simulink model "SuspensionModel"  (R2023a)
settings: Solver=FixedStepAuto  StartTime=0.0  StopTime=30  FixedStep=1e-3  RelTol=1e-3
model workspace (MAT data in the model file):
  A = [0  1  0  -1; -444.444444444  -26.3931623932  0  26.3931623932; 0  0  0  1; 2418.60465116  143.627906977  -9302.3255814  -143.627906977]
  A_eso = [0  1  0; 0  0  1; 0  0  0]
  B = [0  0; 0  0.0042735042735; -1  0; 0  -0.0232558139535]
  B_eso_th = [0; 333.333333333; 0]
  B_eso_y = [0; 0.8; 0]
  C = [1  0  0  0; 0  1  0  0; 0  0  1  0; 0  0  0  1; -444.444444444  -26.3931623932  0  26.3931623932]
  C_eso = [1 0 0]
  D = [0  0; 0  0; 0  0; 0  0; 0  0.0042735042735]
  I = 0.003
  Ic_xnl = [0; 0; 0; 0; 0.349065850399; 0]
  Iyy = 2100
  K = [40277.510375 6943.43713521 -89611.1366666 302.327568335]
  Kd = 5239.23468894
  Kd_2 = 0
  Kd_th = 7.53982236862
  Kd_y = 7.53982236862
  Ki = 3819451.68393
  Ki_2 = 12673.3447819
  Kp = 319533.641021
  Kp_2 = 160
  Kp_th = 14.2122303376
  Kp_y = 14.2122303376
  L = 0.35
  L_eso_th = [56.5486677646; 1065.91727532; 6697.35576294]
  L_eso_y = [56.5486677646; 1065.91727532; 6697.35576294]
  Lf = 0.9
  Lr = 1.2
  Mb = 1200
  Q = [10000000000  0  0  0; 0  100000000  0  0; 0  0  1  0; 0  0  0  1]
  R = 1
  T_f = 5
  b_th = 333.333333333
  b_y = 0.8
  bs = 6176
  bus = 0
  cf = 2000
  cr = 2000
  elapsed_time_simulation = 14.1875694
  fc_th = 0.6
  fc_y = 0.6
  g = 9.81
  h = 0.2
  i = 125
  kf = 28000
  kr = 21000
  ks = 104000
  kus = 400000
  m = 1
  model_sim = Simulink.SimulationOutput
  model_sim.Data.force.Fa_LQR = timeseries
  model_sim.Data.force.Fa_LQR.Name = 'Fa_LQR'
  model_sim.Data.force.Fa_LQR.DataInfo = tsdata.datametadata
  model_sim.Data.force.Fa_LQR.DataInfo.Interpolation = tsdata.interpolation
  model_sim.Data.force.Fa_LQR.DataInfo.Interpolation.Fhandle : function handle (value not decoded)
  model_sim.Data.force.Fa_LQR.DataInfo.Interpolation.Name = 'linear'
  model_sim.Data.force.Fa_LQR.TimeInfo = tsdata.timemetadata
  model_sim.Data.force.Fa_LQR.TimeInfo.Length = 5001
  model_sim.Data.force.Fa_LQR.TimeInfo.DuplicateTimes = 0
  model_sim.Data.force.Fa_LQR.TimeInfo.Increment_ = 0.001
  model_sim.Data.force.Fa_LQR.TimeInfo.Start_ = 0
  model_sim.Data.force.Fa_LQR.TimeInfo.Initialized = 1
  model_sim.Data.force.Fa_LQR.QualityInfo = tsdata.qualmetadata
  model_sim.Data.force.Fa_LQR.Data_ = [0 0 0 0 0 0 0 0 0 0 0 0 ... (5001 elements, 5001x1)]
  model_sim.Data.force.Fa_PID = timeseries
  model_sim.Data.force.Fa_PID.Name = 'Fa_PID'
  model_sim.Data.force.Fa_PID.DataInfo = tsdata.datametadata
  model_sim.Data.force.Fa_PID.DataInfo.Interpolation = tsdata.interpolation
  model_sim.Data.force.Fa_PID.DataInfo.Interpolation.Fhandle : function handle (value not decoded)
  model_sim.Data.force.Fa_PID.DataInfo.Interpolation.Name = 'linear'
  model_sim.Data.force.Fa_PID.TimeInfo = tsdata.timemetadata
  model_sim.Data.force.Fa_PID.TimeInfo.Length = 5001
  model_sim.Data.force.Fa_PID.TimeInfo.DuplicateTimes = 0
  model_sim.Data.force.Fa_PID.TimeInfo.Increment_ = 0.001
  model_sim.Data.force.Fa_PID.TimeInfo.Start_ = 0
  model_sim.Data.force.Fa_PID.TimeInfo.Initialized = 1
  model_sim.Data.force.Fa_PID.QualityInfo = tsdata.qualmetadata
  model_sim.Data.force.Fa_PID.Data_ = [0 0 0 0 0 0 0 0 0 0 0 0 ... (5001 elements, 5001x1)]
  model_sim.Data.force.Fa_passive = timeseries
  model_sim.Data.force.Fa_passive.Name = 'Fa_passive'
  model_sim.Data.force.Fa_passive.DataInfo = tsdata.datametadata
  model_sim.Data.force.Fa_passive.DataInfo.Interpolation = tsdata.interpolation
  model_sim.Data.force.Fa_passive.DataInfo.Interpolation.Fhandle : function handle (value not decoded)
  model_sim.Data.force.Fa_passive.DataInfo.Interpolation.Name = 'zoh'
  model_sim.Data.force.Fa_passive.TimeInfo = tsdata.timemetadata
  model_sim.Data.force.Fa_passive.TimeInfo.Length = 1
  model_sim.Data.force.Fa_passive.TimeInfo.DuplicateTimes = 0
  model_sim.Data.force.Fa_passive.TimeInfo.Time_ = 0
  model_sim.Data.force.Fa_passive.TimeInfo.Initialized = 1
  model_sim.Data.force.Fa_passive.QualityInfo = tsdata.qualmetadata
  model_sim.Data.force.Fa_passive.Data_ = 0
  model_sim.Data.ms_motion.zs_LQR = timeseries
  model_sim.Data.ms_motion.zs_LQR.Name = 'zs_LQR'
  model_sim.Data.ms_motion.zs_LQR.DataInfo = tsdata.datametadata
  model_sim.Data.ms_motion.zs_LQR.DataInfo.Interpolation = tsdata.interpolation
  model_sim.Data.ms_motion.zs_LQR.DataInfo.Interpolation.Fhandle : function handle (value not decoded)
  model_sim.Data.ms_motion.zs_LQR.DataInfo.Interpolation.Name = 'linear'
  model_sim.Data.ms_motion.zs_LQR.TimeInfo = tsdata.timemetadata
  model_sim.Data.ms_motion.zs_LQR.TimeInfo.Length = 5001
  model_sim.Data.ms_motion.zs_LQR.TimeInfo.DuplicateTimes = 0
  model_sim.Data.ms_motion.zs_LQR.TimeInfo.Increment_ = 0.001
  model_sim.Data.ms_motion.zs_LQR.TimeInfo.Start_ = 0
  model_sim.Data.ms_motion.zs_LQR.TimeInfo.Initialized = 1
  model_sim.Data.ms_motion.zs_LQR.QualityInfo = tsdata.qualmetadata
  model_sim.Data.ms_motion.zs_LQR.Data_ = [0 0 0 0 0 0 0 0 0 0 0 0 ... (5001 elements, 5001x1)]
  model_sim.Data.ms_motion.zs_PID = timeseries
  model_sim.Data.ms_motion.zs_PID.Name = 'zs_PID'
  model_sim.Data.ms_motion.zs_PID.DataInfo = tsdata.datametadata
  model_sim.Data.ms_motion.zs_PID.DataInfo.Interpolation = tsdata.interpolation
  model_sim.Data.ms_motion.zs_PID.DataInfo.Interpolation.Fhandle : function handle (value not decoded)
  model_sim.Data.ms_motion.zs_PID.DataInfo.Interpolation.Name = 'linear'
  model_sim.Data.ms_motion.zs_PID.TimeInfo = tsdata.timemetadata
  model_sim.Data.ms_motion.zs_PID.TimeInfo.Length = 5001
  model_sim.Data.ms_motion.zs_PID.TimeInfo.DuplicateTimes = 0
  model_sim.Data.ms_motion.zs_PID.TimeInfo.Increment_ = 0.001
  model_sim.Data.ms_motion.zs_PID.TimeInfo.Start_ = 0
  model_sim.Data.ms_motion.zs_PID.TimeInfo.Initialized = 1
  model_sim.Data.ms_motion.zs_PID.QualityInfo = tsdata.qualmetadata
  model_sim.Data.ms_motion.zs_PID.Data_ = [0 0 0 0 0 0 0 0 0 0 0 0 ... (5001 elements, 5001x1)]
  model_sim.Data.ms_motion.zs_passive = timeseries
  model_sim.Data.ms_motion.zs_passive.Name = 'zs_passive'
  model_sim.Data.ms_motion.zs_passive.DataInfo = tsdata.datametadata
  model_sim.Data.ms_motion.zs_passive.DataInfo.Interpolation = tsdata.interpolation
  model_sim.Data.ms_motion.zs_passive.DataInfo.Interpolation.Fhandle : function handle (value not decoded)
  model_sim.Data.ms_motion.zs_passive.DataInfo.Interpolation.Name = 'linear'
  model_sim.Data.ms_motion.zs_passive.TimeInfo = tsdata.timemetadata
  model_sim.Data.ms_motion.zs_passive.TimeInfo.Length = 5001
  model_sim.Data.ms_motion.zs_passive.TimeInfo.DuplicateTimes = 0
  model_sim.Data.ms_motion.zs_passive.TimeInfo.Increment_ = 0.001
  model_sim.Data.ms_motion.zs_passive.TimeInfo.Start_ = 0
  model_sim.Data.ms_motion.zs_passive.TimeInfo.Initialized = 1
  model_sim.Data.ms_motion.zs_passive.QualityInfo = tsdata.qualmetadata
  model_sim.Data.ms_motion.zs_passive.Data_ = [0 0 0 0 0 0 0 0 0 0 0 0 ... (5001 elements, 5001x1)]
  model_sim.Data.road_profile = timeseries
  model_sim.Data.road_profile.Name = 'zr'
  model_sim.Data.road_profile.DataInfo = tsdata.datametadata
  model_sim.Data.road_profile.DataInfo.Interpolation = tsdata.interpolation
  model_sim.Data.road_profile.DataInfo.Interpolation.Fhandle : function handle (value not decoded)
  model_sim.Data.road_profile.DataInfo.Interpolation.Name = 'linear'
  model_sim.Data.road_profile.TimeInfo = tsdata.timemetadata
  model_sim.Data.road_profile.TimeInfo.Length = 5001
  model_sim.Data.road_profile.TimeInfo.DuplicateTimes = 0
  model_sim.Data.road_profile.TimeInfo.Increment_ = 0.001
  model_sim.Data.road_profile.TimeInfo.Start_ = 0
  model_sim.Data.road_profile.TimeInfo.Initialized = 1
  model_sim.Data.road_profile.QualityInfo = tsdata.qualmetadata
  model_sim.Data.road_profile.Data_ = [0 0 0 0 0 0 0 0 0 0 0 0 ... (5001 elements, 1x1x5001)]
  model_sim.Data.road_profile.IsTimeFirst_ = 0
  model_sim.Data.sprung_mass_acc.zs_dd_PID = timeseries
  model_sim.Data.sprung_mass_acc.zs_dd_PID.Name = 'zs_dd_PID'
  model_sim.Data.sprung_mass_acc.zs_dd_PID.DataInfo = tsdata.datametadata
  model_sim.Data.sprung_mass_acc.zs_dd_PID.DataInfo.Interpolation = tsdata.interpolation
  model_sim.Data.sprung_mass_acc.zs_dd_PID.DataInfo.Interpolation.Fhandle : function handle (value not decoded)
  model_sim.Data.sprung_mass_acc.zs_dd_PID.DataInfo.Interpolation.Name = 'linear'
  model_sim.Data.sprung_mass_acc.zs_dd_PID.TimeInfo = tsdata.timemetadata
  model_sim.Data.sprung_mass_acc.zs_dd_PID.TimeInfo.Length = 5001
  model_sim.Data.sprung_mass_acc.zs_dd_PID.TimeInfo.DuplicateTimes = 0
  model_sim.Data.sprung_mass_acc.zs_dd_PID.TimeInfo.Increment_ = 0.001
  model_sim.Data.sprung_mass_acc.zs_dd_PID.TimeInfo.Start_ = 0
  model_sim.Data.sprung_mass_acc.zs_dd_PID.TimeInfo.Initialized = 1
  model_sim.Data.sprung_mass_acc.zs_dd_PID.QualityInfo = tsdata.qualmetadata
  model_sim.Data.sprung_mass_acc.zs_dd_PID.Data_ = [0 0 0 0 0 0 0 0 0 0 0 0 ... (5001 elements, 5001x1)]
  model_sim.Data.sprung_mass_acc.zs_dd_LQR = timeseries
  model_sim.Data.sprung_mass_acc.zs_dd_LQR.Name = 'zs_dd_LQR'
  model_sim.Data.sprung_mass_acc.zs_dd_LQR.DataInfo = tsdata.datametadata
  model_sim.Data.sprung_mass_acc.zs_dd_LQR.DataInfo.Interpolation = tsdata.interpolation
  model_sim.Data.sprung_mass_acc.zs_dd_LQR.DataInfo.Interpolation.Fhandle : function handle (value not decoded)
  model_sim.Data.sprung_mass_acc.zs_dd_LQR.DataInfo.Interpolation.Name = 'linear'
  model_sim.Data.sprung_mass_acc.zs_dd_LQR.TimeInfo = tsdata.timemetadata
  model_sim.Data.sprung_mass_acc.zs_dd_LQR.TimeInfo.Length = 5001
  model_sim.Data.sprung_mass_acc.zs_dd_LQR.TimeInfo.DuplicateTimes = 0
  model_sim.Data.sprung_mass_acc.zs_dd_LQR.TimeInfo.Increment_ = 0.001
  model_sim.Data.sprung_mass_acc.zs_dd_LQR.TimeInfo.Start_ = 0
  model_sim.Data.sprung_mass_acc.zs_dd_LQR.TimeInfo.Initialized = 1
  model_sim.Data.sprung_mass_acc.zs_dd_LQR.QualityInfo = tsdata.qualmetadata
  model_sim.Data.sprung_mass_acc.zs_dd_LQR.Data_ = [0 0 0 0 0 0 0 0 0 0 0 0 ... (5001 elements, 5001x1)]
  model_sim.Data.sprung_mass_acc.zs_dd_passive = timeseries
  model_sim.Data.sprung_mass_acc.zs_dd_passive.Name = 'zs_dd_passive'
  model_sim.Data.sprung_mass_acc.zs_dd_passive.DataInfo = tsdata.datametadata
  model_sim.Data.sprung_mass_acc.zs_dd_passive.DataInfo.Interpolation = tsdata.interpolation
  model_sim.Data.sprung_mass_acc.zs_dd_passive.DataInfo.Interpolation.Fhandle : function handle (value not decoded)
  model_sim.Data.sprung_mass_acc.zs_dd_passive.DataInfo.Interpolation.Name = 'linear'
  model_sim.Data.sprung_mass_acc.zs_dd_passive.TimeInfo = tsdata.timemetadata
  model_sim.Data.sprung_mass_acc.zs_dd_passive.TimeInfo.Length = 5001
  model_sim.Data.sprung_mass_acc.zs_dd_passive.TimeInfo.DuplicateTimes = 0
  model_sim.Data.sprung_mass_acc.zs_dd_passive.TimeInfo.Increment_ = 0.001
  model_sim.Data.sprung_mass_acc.zs_dd_passive.TimeInfo.Start_ = 0
  model_sim.Data.sprung_mass_acc.zs_dd_passive.TimeInfo.Initialized = 1
  model_sim.Data.sprung_mass_acc.zs_dd_passive.QualityInfo = tsdata.qualmetadata
  model_sim.Data.sprung_mass_acc.zs_dd_passive.Data_ = [0 0 0 0 0 0 0 0 0 0 0 0 ... (5001 elements, 5001x1)]
  model_sim.Data.state.state_PID.zs_zus = timeseries
  model_sim.Data.state.state_PID.zs_zus.Name = 'zs_zus'
  model_sim.Data.state.state_PID.zs_zus.DataInfo = tsdata.datametadata
  model_sim.Data.state.state_PID.zs_zus.DataInfo.Interpolation = tsdata.interpolation
  model_sim.Data.state.state_PID.zs_zus.DataInfo.Interpolation.Fhandle : function handle (value not decoded)
  model_sim.Data.state.state_PID.zs_zus.DataInfo.Interpolation.Name = 'linear'
  model_sim.Data.state.state_PID.zs_zus.TimeInfo = tsdata.timemetadata
  model_sim.Data.state.state_PID.zs_zus.TimeInfo.Length = 5001
  model_sim.Data.state.state_PID.zs_zus.TimeInfo.DuplicateTimes = 0
  model_sim.Data.state.state_PID.zs_zus.TimeInfo.Increment_ = 0.001
  model_sim.Data.state.state_PID.zs_zus.TimeInfo.Start_ = 0
  model_sim.Data.state.state_PID.zs_zus.TimeInfo.Initialized = 1
  model_sim.Data.state.state_PID.zs_zus.QualityInfo = tsdata.qualmetadata
  model_sim.Data.state.state_PID.zs_zus.Data_ = [0 0 0 0 0 0 0 0 0 0 0 0 ... (5001 elements, 5001x1)]
  model_sim.Data.state.state_PID.zs_d = timeseries
  model_sim.Data.state.state_PID.zs_d.Name = 'zs_d'
  model_sim.Data.state.state_PID.zs_d.DataInfo = tsdata.datametadata
  model_sim.Data.state.state_PID.zs_d.DataInfo.Interpolation = tsdata.interpolation
  model_sim.Data.state.state_PID.zs_d.DataInfo.Interpolation.Fhandle : function handle (value not decoded)
  model_sim.Data.state.state_PID.zs_d.DataInfo.Interpolation.Name = 'linear'
  model_sim.Data.state.state_PID.zs_d.TimeInfo = tsdata.timemetadata
  model_sim.Data.state.state_PID.zs_d.TimeInfo.Length = 5001
  model_sim.Data.state.state_PID.zs_d.TimeInfo.DuplicateTimes = 0
  model_sim.Data.state.state_PID.zs_d.TimeInfo.Increment_ = 0.001
  model_sim.Data.state.state_PID.zs_d.TimeInfo.Start_ = 0
  model_sim.Data.state.state_PID.zs_d.TimeInfo.Initialized = 1
  model_sim.Data.state.state_PID.zs_d.QualityInfo = tsdata.qualmetadata
  model_sim.Data.state.state_PID.zs_d.Data_ = [0 0 0 0 0 0 0 0 0 0 0 0 ... (5001 elements, 5001x1)]
  model_sim.Data.state.state_PID.zus_zr = timeseries
  model_sim.Data.state.state_PID.zus_zr.Name = 'zus_zr'
  model_sim.Data.state.state_PID.zus_zr.DataInfo = tsdata.datametadata
  model_sim.Data.state.state_PID.zus_zr.DataInfo.Interpolation = tsdata.interpolation
  model_sim.Data.state.state_PID.zus_zr.DataInfo.Interpolation.Fhandle : function handle (value not decoded)
  model_sim.Data.state.state_PID.zus_zr.DataInfo.Interpolation.Name = 'linear'
  model_sim.Data.state.state_PID.zus_zr.TimeInfo = tsdata.timemetadata
  model_sim.Data.state.state_PID.zus_zr.TimeInfo.Length = 5001
  model_sim.Data.state.state_PID.zus_zr.TimeInfo.DuplicateTimes = 0
  model_sim.Data.state.state_PID.zus_zr.TimeInfo.Increment_ = 0.001
  model_sim.Data.state.state_PID.zus_zr.TimeInfo.Start_ = 0
  model_sim.Data.state.state_PID.zus_zr.TimeInfo.Initialized = 1
  model_sim.Data.state.state_PID.zus_zr.QualityInfo = tsdata.qualmetadata
  model_sim.Data.state.state_PID.zus_zr.Data_ = [0 0 0 0 0 0 0 0 0 0 0 0 ... (5001 elements, 5001x1)]
  model_sim.Data.state.state_PID.zus_d = timeseries
  model_sim.Data.state.state_PID.zus_d.Name = 'zus_d'
  model_sim.Data.state.state_PID.zus_d.DataInfo = tsdata.datametadata
  model_sim.Data.state.state_PID.zus_d.DataInfo.Interpolation = tsdata.interpolation
  model_sim.Data.state.state_PID.zus_d.DataInfo.Interpolation.Fhandle : function handle (value not decoded)
  model_sim.Data.state.state_PID.zus_d.DataInfo.Interpolation.Name = 'linear'
  model_sim.Data.state.state_PID.zus_d.TimeInfo = tsdata.timemetadata
  model_sim.Data.state.state_PID.zus_d.TimeInfo.Length = 5001
  model_sim.Data.state.state_PID.zus_d.TimeInfo.DuplicateTimes = 0
  model_sim.Data.state.state_PID.zus_d.TimeInfo.Increment_ = 0.001
  model_sim.Data.state.state_PID.zus_d.TimeInfo.Start_ = 0
  model_sim.Data.state.state_PID.zus_d.TimeInfo.Initialized = 1
  model_sim.Data.state.state_PID.zus_d.QualityInfo = tsdata.qualmetadata
  model_sim.Data.state.state_PID.zus_d.Data_ = [0 0 0 0 0 0 0 0 0 0 0 0 ... (5001 elements, 5001x1)]
  model_sim.Data.state.state_LQR.zs_zus = timeseries
  model_sim.Data.state.state_LQR.zs_zus.Name = 'zs_zus'
  model_sim.Data.state.state_LQR.zs_zus.DataInfo = tsdata.datametadata
  model_sim.Data.state.state_LQR.zs_zus.DataInfo.Interpolation = tsdata.interpolation
  model_sim.Data.state.state_LQR.zs_zus.DataInfo.Interpolation.Fhandle : function handle (value not decoded)
  model_sim.Data.state.state_LQR.zs_zus.DataInfo.Interpolation.Name = 'linear'
  model_sim.Data.state.state_LQR.zs_zus.TimeInfo = tsdata.timemetadata
  model_sim.Data.state.state_LQR.zs_zus.TimeInfo.Length = 5001
  model_sim.Data.state.state_LQR.zs_zus.TimeInfo.DuplicateTimes = 0
  model_sim.Data.state.state_LQR.zs_zus.TimeInfo.Increment_ = 0.001
  model_sim.Data.state.state_LQR.zs_zus.TimeInfo.Start_ = 0
  model_sim.Data.state.state_LQR.zs_zus.TimeInfo.Initialized = 1
  model_sim.Data.state.state_LQR.zs_zus.QualityInfo = tsdata.qualmetadata
  model_sim.Data.state.state_LQR.zs_zus.Data_ = [0 0 0 0 0 0 0 0 0 0 0 0 ... (5001 elements, 5001x1)]
  model_sim.Data.state.state_LQR.zs_d = timeseries
  model_sim.Data.state.state_LQR.zs_d.Name = 'zs_d'
  model_sim.Data.state.state_LQR.zs_d.DataInfo = tsdata.datametadata
  model_sim.Data.state.state_LQR.zs_d.DataInfo.Interpolation = tsdata.interpolation
  model_sim.Data.state.state_LQR.zs_d.DataInfo.Interpolation.Fhandle : function handle (value not decoded)
  model_sim.Data.state.state_LQR.zs_d.DataInfo.Interpolation.Name = 'linear'
  model_sim.Data.state.state_LQR.zs_d.TimeInfo = tsdata.timemetadata
  model_sim.Data.state.state_LQR.zs_d.TimeInfo.Length = 5001
  model_sim.Data.state.state_LQR.zs_d.TimeInfo.DuplicateTimes = 0
  model_sim.Data.state.state_LQR.zs_d.TimeInfo.Increment_ = 0.001
  model_sim.Data.state.state_LQR.zs_d.TimeInfo.Start_ = 0
  model_sim.Data.state.state_LQR.zs_d.TimeInfo.Initialized = 1
  model_sim.Data.state.state_LQR.zs_d.QualityInfo = tsdata.qualmetadata
  model_sim.Data.state.state_LQR.zs_d.Data_ = [0 0 0 0 0 0 0 0 0 0 0 0 ... (5001 elements, 5001x1)]
  model_sim.Data.state.state_LQR.zus_zr = timeseries
  model_sim.Data.state.state_LQR.zus_zr.Name = 'zus_zr'
  model_sim.Data.state.state_LQR.zus_zr.DataInfo = tsdata.datametadata
  model_sim.Data.state.state_LQR.zus_zr.DataInfo.Interpolation = tsdata.interpolation
  model_sim.Data.state.state_LQR.zus_zr.DataInfo.Interpolation.Fhandle : function handle (value not decoded)
  model_sim.Data.state.state_LQR.zus_zr.DataInfo.Interpolation.Name = 'linear'
  model_sim.Data.state.state_LQR.zus_zr.TimeInfo = tsdata.timemetadata
  model_sim.Data.state.state_LQR.zus_zr.TimeInfo.Length = 5001
  model_sim.Data.state.state_LQR.zus_zr.TimeInfo.DuplicateTimes = 0
  model_sim.Data.state.state_LQR.zus_zr.TimeInfo.Increment_ = 0.001
  model_sim.Data.state.state_LQR.zus_zr.TimeInfo.Start_ = 0
  model_sim.Data.state.state_LQR.zus_zr.TimeInfo.Initialized = 1
  model_sim.Data.state.state_LQR.zus_zr.QualityInfo = tsdata.qualmetadata
  model_sim.Data.state.state_LQR.zus_zr.Data_ = [0 0 0 0 0 0 0 0 0 0 0 0 ... (5001 elements, 5001x1)]
  model_sim.Data.state.state_LQR.zus_d = timeseries
  model_sim.Data.state.state_LQR.zus_d.Name = 'zus_d'
  model_sim.Data.state.state_LQR.zus_d.DataInfo = tsdata.datametadata
  model_sim.Data.state.state_LQR.zus_d.DataInfo.Interpolation = tsdata.interpolation
  model_sim.Data.state.state_LQR.zus_d.DataInfo.Interpolation.Fhandle : function handle (value not decoded)
  model_sim.Data.state.state_LQR.zus_d.DataInfo.Interpolation.Name = 'linear'
  model_sim.Data.state.state_LQR.zus_d.TimeInfo = tsdata.timemetadata
  model_sim.Data.state.state_LQR.zus_d.TimeInfo.Length = 5001
  model_sim.Data.state.state_LQR.zus_d.TimeInfo.DuplicateTimes = 0
  model_sim.Data.state.state_LQR.zus_d.TimeInfo.Increment_ = 0.001
  model_sim.Data.state.state_LQR.zus_d.TimeInfo.Start_ = 0
  model_sim.Data.state.state_LQR.zus_d.TimeInfo.Initialized = 1
  model_sim.Data.state.state_LQR.zus_d.QualityInfo = tsdata.qualmetadata
  model_sim.Data.state.state_LQR.zus_d.Data_ = [0 0 0 0 0 0 0 0 0 0 0 0 ... (5001 elements, 5001x1)]
  model_sim.Data.state.state_passive.zs_zus = timeseries
  model_sim.Data.state.state_passive.zs_zus.Name = 'zs_zus'
  model_sim.Data.state.state_passive.zs_zus.DataInfo = tsdata.datametadata
  model_sim.Data.state.state_passive.zs_zus.DataInfo.Interpolation = tsdata.interpolation
  model_sim.Data.state.state_passive.zs_zus.DataInfo.Interpolation.Fhandle : function handle (value not decoded)
  model_sim.Data.state.state_passive.zs_zus.DataInfo.Interpolation.Name = 'linear'
  model_sim.Data.state.state_passive.zs_zus.TimeInfo = tsdata.timemetadata
  model_sim.Data.state.state_passive.zs_zus.TimeInfo.Length = 5001
  model_sim.Data.state.state_passive.zs_zus.TimeInfo.DuplicateTimes = 0
  model_sim.Data.state.state_passive.zs_zus.TimeInfo.Increment_ = 0.001
  model_sim.Data.state.state_passive.zs_zus.TimeInfo.Start_ = 0
  model_sim.Data.state.state_passive.zs_zus.TimeInfo.Initialized = 1
  model_sim.Data.state.state_passive.zs_zus.QualityInfo = tsdata.qualmetadata
  model_sim.Data.state.state_passive.zs_zus.Data_ = [0 0 0 0 0 0 0 0 0 0 0 0 ... (5001 elements, 5001x1)]
  model_sim.Data.state.state_passive.zs_d = timeseries
  model_sim.Data.state.state_passive.zs_d.Name = 'zs_d'
  model_sim.Data.state.state_passive.zs_d.DataInfo = tsdata.datametadata
  model_sim.Data.state.state_passive.zs_d.DataInfo.Interpolation = tsdata.interpolation
  model_sim.Data.state.state_passive.zs_d.DataInfo.Interpolation.Fhandle : function handle (value not decoded)
  model_sim.Data.state.state_passive.zs_d.DataInfo.Interpolation.Name = 'linear'
  model_sim.Data.state.state_passive.zs_d.TimeInfo = tsdata.timemetadata
  model_sim.Data.state.state_passive.zs_d.TimeInfo.Length = 5001
  model_sim.Data.state.state_passive.zs_d.TimeInfo.DuplicateTimes = 0
  model_sim.Data.state.state_passive.zs_d.TimeInfo.Increment_ = 0.001
  model_sim.Data.state.state_passive.zs_d.TimeInfo.Start_ = 0
  model_sim.Data.state.state_passive.zs_d.TimeInfo.Initialized = 1
  model_sim.Data.state.state_passive.zs_d.QualityInfo = tsdata.qualmetadata
  model_sim.Data.state.state_passive.zs_d.Data_ = [0 0 0 0 0 0 0 0 0 0 0 0 ... (5001 elements, 5001x1)]
  model_sim.Data.state.state_passive.zus_zr = timeseries
  model_sim.Data.state.state_passive.zus_zr.Name = 'zus_zr'
  model_sim.Data.state.state_passive.zus_zr.DataInfo = tsdata.datametadata
  model_sim.Data.state.state_passive.zus_zr.DataInfo.Interpolation = tsdata.interpolation
  model_sim.Data.state.state_passive.zus_zr.DataInfo.Interpolation.Fhandle : function handle (value not decoded)
  model_sim.Data.state.state_passive.zus_zr.DataInfo.Interpolation.Name = 'linear'
  model_sim.Data.state.state_passive.zus_zr.TimeInfo = tsdata.timemetadata
  model_sim.Data.state.state_passive.zus_zr.TimeInfo.Length = 5001
  model_sim.Data.state.state_passive.zus_zr.TimeInfo.DuplicateTimes = 0
  model_sim.Data.state.state_passive.zus_zr.TimeInfo.Increment_ = 0.001
  model_sim.Data.state.state_passive.zus_zr.TimeInfo.Start_ = 0
  model_sim.Data.state.state_passive.zus_zr.TimeInfo.Initialized = 1
  model_sim.Data.state.state_passive.zus_zr.QualityInfo = tsdata.qualmetadata
  model_sim.Data.state.state_passive.zus_zr.Data_ = [0 0 0 0 0 0 0 0 0 0 0 0 ... (5001 elements, 5001x1)]
  model_sim.Data.state.state_passive.zus_d = timeseries
  model_sim.Data.state.state_passive.zus_d.Name = 'zus_d'
  model_sim.Data.state.state_passive.zus_d.DataInfo = tsdata.datametadata
  model_sim.Data.state.state_passive.zus_d.DataInfo.Interpolation = tsdata.interpolation
  model_sim.Data.state.state_passive.zus_d.DataInfo.Interpolation.Fhandle : function handle (value not decoded)
  model_sim.Data.state.state_passive.zus_d.DataInfo.Interpolation.Name = 'linear'
  model_sim.Data.state.state_passive.zus_d.TimeInfo = tsdata.timemetadata
  model_sim.Data.state.state_passive.zus_d.TimeInfo.Length = 5001
  model_sim.Data.state.state_passive.zus_d.TimeInfo.DuplicateTimes = 0
  model_sim.Data.state.state_passive.zus_d.TimeInfo.Increment_ = 0.001
  model_sim.Data.state.state_passive.zus_d.TimeInfo.Start_ = 0
  model_sim.Data.state.state_passive.zus_d.TimeInfo.Initialized = 1
  model_sim.Data.state.state_passive.zus_d.QualityInfo = tsdata.qualmetadata
  model_sim.Data.state.state_passive.zus_d.Data_ = [0 0 0 0 0 0 0 0 0 0 0 0 ... (5001 elements, 5001x1)]
  model_sim.Data.tout = [0 0.001 0.002 0.003 0.004 0.005 0.006 0.007 0.008 0.009 0.01 0.011 ... (5001 elements, 5001x1)]
  model_sim.Metadata = Simulink.SimulationMetadata
  model_sim.Metadata.ModelInfo.ModelName = 'Quarter_Car_Suspension_Simulink'
  model_sim.Metadata.ModelInfo.ModelVersion = '2.0'
  model_sim.Metadata.ModelInfo.ModelFilePath = 'C:\Users\omert\Documents\MATLAB\Quarter_Car_Suspension_Simulink.slx'
  model_sim.Metadata.ModelInfo.UserID = 'omert'
  model_sim.Metadata.ModelInfo.MachineName = 'DESKTOP-823S3D7'
  model_sim.Metadata.ModelInfo.Platform = 'PCWIN64'
  model_sim.Metadata.ModelInfo.ModelStructuralChecksum = [3113813742; 4073628985; 3971547785; 3559641876]
  model_sim.Metadata.ModelInfo.SimulationMode = 'normal'
  model_sim.Metadata.ModelInfo.StartTime = 0
  model_sim.Metadata.ModelInfo.StopTime = 5
  model_sim.Metadata.ModelInfo.SolverInfo.Type = 'Fixed-Step'
  model_sim.Metadata.ModelInfo.SolverInfo.Solver = 'ode1'
  model_sim.Metadata.ModelInfo.SolverInfo.FixedStepSize = 0.001
  model_sim.Metadata.ModelInfo.SimulinkVersion.Name = 'Simulink'
  model_sim.Metadata.ModelInfo.SimulinkVersion.Version = '10.7'
  model_sim.Metadata.ModelInfo.SimulinkVersion.Release = '(R2023a)'
  model_sim.Metadata.ModelInfo.SimulinkVersion.Date = '19-Nov-2022'
  model_sim.Metadata.ModelInfo.LoggingInfo.LoggingToFile = 'off'
  model_sim.Metadata.TimingInfo.WallClockTimestampStart = '2023-08-10 00:55:11'
  model_sim.Metadata.TimingInfo.WallClockTimestampStop = '2023-08-10 00:55:25'
  model_sim.Metadata.TimingInfo.InitializationElapsedWallTime = 13.421691
  model_sim.Metadata.TimingInfo.ExecutionElapsedWallTime = 0.1563724
  model_sim.Metadata.TimingInfo.TerminationElapsedWallTime = 0.5363111
  model_sim.Metadata.TimingInfo.TotalElapsedWallTime = 14.1143745
  model_sim.Metadata.TimingInfo.ProfilerData = 'Profiler is not enabled'
  model_sim.Metadata.ExecutionInfo.StopEvent = 'ReachedStopTime'
  model_sim.Metadata.ExecutionInfo.StopEventSource = []
  model_sim.Metadata.ExecutionInfo.StopEventDescription = 'Reached stop time of 5'
  model_sim.Metadata.ExecutionInfo.ErrorDiagnostic = []
  model_sim.Metadata.ExecutionInfo.WarningDiagnostics(1).Diagnostic = MSLDiagnostic
  model_sim.Metadata.ExecutionInfo.WarningDiagnostics(1).Diagnostic.identifier = 'Simulink:Engine:WarnAlgLoopsFound'
  model_sim.Metadata.ExecutionInfo.WarningDiagnostics(1).Diagnostic.message = 'Block diagram ''<a href="matlab:open_system (''Quarter_Car_Suspension_Simulink'')">Quarter_Car_Suspension_Simulink</a>'' contains 2 algebraic loop(s). To see more details about the loops use the command <a href="matlab:Simulink.BlockDiagram.getAlgebraicLoops(bdroot);">Simulink.BlockDiagram.getAlgebraicLoops(''Quarter_Car_Suspension_Simulink'') </a> or the command line Simulink debugger by typing <a href="matlab:sldebug(bdroot);">sldebug(''Quarter_Car_Suspension_Simulink'') </a> in the MATLAB command window. To eliminate this message, set <a href="matlab:configset.internal.open(''Quarter_Car_Suspension_Simulink'',''AlgebraicLoopMsg'');">Algebraic loop</a> to "none".'
  model_sim.Metadata.ExecutionInfo.WarningDiagnostics(1).Diagnostic.paths = {'Quarter_Car_Suspension_Simulink'}
  model_sim.Metadata.ExecutionInfo.WarningDiagnostics(1).Diagnostic.arguments = {'Quarter_Car_Suspension_Simulink', 2, 'Quarter_Car_Suspension_Simulink', 'Quarter_Car_Suspension_Simulink'}
  model_sim.Metadata.ExecutionInfo.WarningDiagnostics(1).Diagnostic.stack = struct([])
  model_sim.Metadata.ExecutionInfo.WarningDiagnostics(1).Diagnostic.priority = 2
  model_sim.Metadata.ExecutionInfo.WarningDiagnostics(1).SimulationPhase = 'Initialization'
  model_sim.Metadata.ExecutionInfo.WarningDiagnostics(1).SimulationTime = []
  model_sim.Metadata.ExecutionInfo.WarningDiagnostics(2).Diagnostic = MSLDiagnostic
  model_sim.Metadata.ExecutionInfo.WarningDiagnostics(2).Diagnostic.identifier = 'Simulink:Engine:SortDiscontinuityInAlgLoop'
  model_sim.Metadata.ExecutionInfo.WarningDiagnostics(2).Diagnostic.message = 'Discontinuities detected within algebraic loop(s), may have trouble solving'
  model_sim.Metadata.ExecutionInfo.WarningDiagnostics(2).Diagnostic.stack = struct([])
  model_sim.Metadata.ExecutionInfo.WarningDiagnostics(2).Diagnostic.priority = 2
  model_sim.Metadata.ExecutionInfo.WarningDiagnostics(2).SimulationPhase = 'Initialization'
  model_sim.Metadata.ExecutionInfo.WarningDiagnostics(2).SimulationTime = []
  model_sim.Metadata.AppInfo = struct()
  ms = 234
  mus = 43
  pid = pid
  pid.IOSize_ = [1 1]
  pid.Data_ = ltipack.piddataP
  pid.Data_.Delay.Input = 0
  pid.Data_.Delay.Output = 0
  pid.Data_.Delay.IO = 0
  pid.Data_.Ts = 0
  pid.Data_.Kp = 219533.641021
  pid.Data_.Ki = 1819451.68393
  pid.Data_.Kd = 5139.23468894
  pid.Data_.Tf = 0
  pid_2 = pid
  pid_2.IOSize_ = [1 1]
  pid_2.Data_ = ltipack.piddataP
  pid_2.Data_.Delay.Input = 0
  pid_2.Data_.Delay.Output = 0
  pid_2.Data_.Delay.IO = 0
  pid_2.Data_.Ts = 0
  pid_2.Data_.Kp = 0
  pid_2.Data_.Ki = 6673.34478191
  pid_2.Data_.Kd = 0
  pid_2.Data_.Tf = 0
  qcar = ss
  qcar.InputName_ = ["zr_d"; "Fa"]
  qcar.OutputName_ = ["zs-zus"; "zs_dot"; "zus-zr"; "zus_dot"; "zs_dotdot"]
  qcar.IOSize_ = [5 2]
  qcar.Data_ = ltipack.ssdata
  qcar.Data_.StateName = ["zs-zus (m)"; "zs_dot (m/s)"; "zus-zr (m)"; "zus_dot (m/s)"]
  qcar.Data_.a = [0  1  0  -1; -444.444444444  -26.3931623932  0  26.3931623932; 0  0  0  1; 2418.60465116  143.627906977  -9302.3255814  -143.627906977]
  qcar.Data_.b = [0  0; 0  0.0042735042735; -1  0; 0  -0.0232558139535]
  qcar.Data_.c = [1  0  0  0; 0  1  0  0; 0  0  1  0; 0  0  0  1; -444.444444444  -26.3931623932  0  26.3931623932]
  qcar.Data_.d = [0  0; 0  0; 0  0; 0  0; 0  0.0042735042735]
  qcar.Data_.Delay.Input = [0; 0]
  qcar.Data_.Delay.Output = [0; 0; 0; 0; 0]
  qcar.Data_.Delay.Internal = []
  qcar.Data_.Ts = 0
  road = 3
  road_profile = timeseries
  road_profile.Name = 'zr'
  road_profile.DataInfo = tsdata.datametadata
  road_profile.DataInfo.Interpolation = tsdata.interpolation
  road_profile.DataInfo.Interpolation.Fhandle : function handle (value not decoded)
  road_profile.DataInfo.Interpolation.Name = 'linear'
  road_profile.TimeInfo = tsdata.timemetadata
  road_profile.TimeInfo.Length = 5001
  road_profile.TimeInfo.DuplicateTimes = 0
  road_profile.TimeInfo.Increment_ = 0.001
  road_profile.TimeInfo.Start_ = 0
  road_profile.TimeInfo.Initialized = 1
  road_profile.QualityInfo = tsdata.qualmetadata
  road_profile.Data_ = [0 0 0 0 0 0 0 0 0 0 0 0 ... (5001 elements, 1x1x5001)]
  road_profile.IsTimeFirst_ = 0
  road_surface = timeseries
  road_surface.Name = 'unnamed'
  road_surface.DataInfo = tsdata.datametadata
  road_surface.DataInfo.Interpolation = tsdata.interpolation
  road_surface.DataInfo.Interpolation.Fhandle : function handle (value not decoded)
  road_surface.DataInfo.Interpolation.Name = 'linear'
  road_surface.TimeInfo = tsdata.timemetadata
  road_surface.TimeInfo.Length = 125
  road_surface.TimeInfo.DuplicateTimes = 0
  road_surface.TimeInfo.Time_ = [0.01; 0.05; 0.09; 0.13; 0.17; 0.21; 0.25; 0.29; 0.33; 0.37; 0.41; 0.45; 0.49; 0.53; 0.57; 0.61; 0.65; 0.69; 0.73; 0.77; 0.81; 0.85; 0.89; 0.93; 0.97; 1.01; 1.05; 1.09; 1.13; 1.17; 1.21; 1.25; 1.29; 1.33; 1.37; 1.41; 1.45; 1.49; 1.53; 1.57; 1.61; 1.65; 1.69; 1.73; 1.77; 1.81; 1.85; 1.89; 1.93; 1.97; 2.01; 2.05; 2.09; 2.13; 2.17; 2.21; 2.25; 2.29; 2.33; 2.37; 2.41; 2.45; 2.49; 2.53; 2.57; 2.61; 2.65; 2.69; 2.73; 2.77; 2.81; 2.85; 2.89; 2.93; 2.97; 3.01; 3.05; 3.09; 3.13; 3.17; 3.21; 3.25; 3.29; 3.33; 3.37; 3.41; 3.45; 3.49; 3.53; 3.57; 3.61; 3.65; 3.69; 3.73; 3.77; 3.81; 3.85; 3.89; 3.93; 3.97; 4.01; 4.05; 4.09; 4.13; 4.17; 4.21; 4.25; 4.29; 4.33; 4.37; 4.41; 4.45; 4.49; 4.53; 4.57; 4.61; 4.65; 4.69; 4.73; 4.77; 4.81; 4.85; 4.89; 4.93; 4.97]
  road_surface.TimeInfo.Initialized = 1
  road_surface.QualityInfo = tsdata.qualmetadata
  road_surface.Data_ = reshape([0 0 0 0 0 0 0 0 0 0 0 0 0 0 0 0 0 0 0 0 0 0 0 0 0 0.0790366704775 0 0 0 0 0 0 0 0 0 0 0 0 0 0 0 0 0 0 0 0 0 0 0 0 0 0 0 0 0 0 0 0 0 0 0 0 0 0 0 0 0 0 0 0 0 0 0 0 0 0 0 0 0 0 0 0 0 0 0 0 0 0 0 0 0 0 0 0 0 0 0 0 0 0 0 0 0 0 0 0 0 0 0 0 0 0 0 0 0 0 0 0 0 0 0 0 0 0 0], [1 1 125])
  sim_time = [0.01 0.05 0.09 0.13 0.17 0.21 0.25 0.29 0.33 0.37 0.41 0.45 0.49 0.53 0.57 0.61 0.65 0.69 0.73 0.77 0.81 0.85 0.89 0.93 0.97 1.01 1.05 1.09 1.13 1.17 1.21 1.25 1.29 1.33 1.37 1.41 1.45 1.49 1.53 1.57 1.61 1.65 1.69 1.73 1.77 1.81 1.85 1.89 1.93 1.97 2.01 2.05 2.09 2.13 2.17 2.21 2.25 2.29 2.33 2.37 2.41 2.45 2.49 2.53 2.57 2.61 2.65 2.69 2.73 2.77 2.81 2.85 2.89 2.93 2.97 3.01 3.05 3.09 3.13 3.17 3.21 3.25 3.29 3.33 3.37 3.41 3.45 3.49 3.53 3.57 3.61 3.65 3.69 3.73 3.77 3.81 3.85 3.89 3.93 3.97 4.01 4.05 4.09 4.13 4.17 4.21 4.25 4.29 4.33 4.37 4.41 4.45 4.49 4.53 4.57 4.61 4.65 4.69 4.73 4.77 4.81 4.85 4.89 4.93 4.97]
  sprung_mass_a.zs_dd_PID = timeseries
  sprung_mass_a.zs_dd_PID.Name = 'zs_dd_PID'
  sprung_mass_a.zs_dd_PID.DataInfo = tsdata.datametadata
  sprung_mass_a.zs_dd_PID.DataInfo.Interpolation = tsdata.interpolation
  sprung_mass_a.zs_dd_PID.DataInfo.Interpolation.Fhandle : function handle (value not decoded)
  sprung_mass_a.zs_dd_PID.DataInfo.Interpolation.Name = 'linear'
  sprung_mass_a.zs_dd_PID.TimeInfo = tsdata.timemetadata
  sprung_mass_a.zs_dd_PID.TimeInfo.Length = 5001
  sprung_mass_a.zs_dd_PID.TimeInfo.DuplicateTimes = 0
  sprung_mass_a.zs_dd_PID.TimeInfo.Increment_ = 0.001
  sprung_mass_a.zs_dd_PID.TimeInfo.Start_ = 0
  sprung_mass_a.zs_dd_PID.TimeInfo.Initialized = 1
  sprung_mass_a.zs_dd_PID.QualityInfo = tsdata.qualmetadata
  sprung_mass_a.zs_dd_PID.Data_ = [0 0 0 0 0 0 0 0 0 0 0 0 ... (5001 elements, 5001x1)]
  sprung_mass_a.zs_dd_LQR = timeseries
  sprung_mass_a.zs_dd_LQR.Name = 'zs_dd_LQR'
  sprung_mass_a.zs_dd_LQR.DataInfo = tsdata.datametadata
  sprung_mass_a.zs_dd_LQR.DataInfo.Interpolation = tsdata.interpolation
  sprung_mass_a.zs_dd_LQR.DataInfo.Interpolation.Fhandle : function handle (value not decoded)
  sprung_mass_a.zs_dd_LQR.DataInfo.Interpolation.Name = 'linear'
  sprung_mass_a.zs_dd_LQR.TimeInfo = tsdata.timemetadata
  sprung_mass_a.zs_dd_LQR.TimeInfo.Length = 5001
  sprung_mass_a.zs_dd_LQR.TimeInfo.DuplicateTimes = 0
  sprung_mass_a.zs_dd_LQR.TimeInfo.Increment_ = 0.001
  sprung_mass_a.zs_dd_LQR.TimeInfo.Start_ = 0
  sprung_mass_a.zs_dd_LQR.TimeInfo.Initialized = 1
  sprung_mass_a.zs_dd_LQR.QualityInfo = tsdata.qualmetadata
  sprung_mass_a.zs_dd_LQR.Data_ = [0 0 0 0 0 0 0 0 0 0 0 0 ... (5001 elements, 5001x1)]
  sprung_mass_a.zs_dd_passive = timeseries
  sprung_mass_a.zs_dd_passive.Name = 'zs_dd_passive'
  sprung_mass_a.zs_dd_passive.DataInfo = tsdata.datametadata
  sprung_mass_a.zs_dd_passive.DataInfo.Interpolation = tsdata.interpolation
  sprung_mass_a.zs_dd_passive.DataInfo.Interpolation.Fhandle : function handle (value not decoded)
  sprung_mass_a.zs_dd_passive.DataInfo.Interpolation.Name = 'linear'
  sprung_mass_a.zs_dd_passive.TimeInfo = tsdata.timemetadata
  sprung_mass_a.zs_dd_passive.TimeInfo.Length = 5001
  sprung_mass_a.zs_dd_passive.TimeInfo.DuplicateTimes = 0
  sprung_mass_a.zs_dd_passive.TimeInfo.Increment_ = 0.001
  sprung_mass_a.zs_dd_passive.TimeInfo.Start_ = 0
  sprung_mass_a.zs_dd_passive.TimeInfo.Initialized = 1
  sprung_mass_a.zs_dd_passive.QualityInfo = tsdata.qualmetadata
  sprung_mass_a.zs_dd_passive.Data_ = [0 0 0 0 0 0 0 0 0 0 0 0 ... (5001 elements, 5001x1)]
  sprung_mass_motion.zs_LQR = timeseries
  sprung_mass_motion.zs_LQR.Name = 'zs_LQR'
  sprung_mass_motion.zs_LQR.DataInfo = tsdata.datametadata
  sprung_mass_motion.zs_LQR.DataInfo.Interpolation = tsdata.interpolation
  sprung_mass_motion.zs_LQR.DataInfo.Interpolation.Fhandle : function handle (value not decoded)
  sprung_mass_motion.zs_LQR.DataInfo.Interpolation.Name = 'linear'
  sprung_mass_motion.zs_LQR.TimeInfo = tsdata.timemetadata
  sprung_mass_motion.zs_LQR.TimeInfo.Length = 5001
  sprung_mass_motion.zs_LQR.TimeInfo.DuplicateTimes = 0
  sprung_mass_motion.zs_LQR.TimeInfo.Increment_ = 0.001
  sprung_mass_motion.zs_LQR.TimeInfo.Start_ = 0
  sprung_mass_motion.zs_LQR.TimeInfo.Initialized = 1
  sprung_mass_motion.zs_LQR.QualityInfo = tsdata.qualmetadata
  sprung_mass_motion.zs_LQR.Data_ = [0 0 0 0 0 0 0 0 0 0 0 0 ... (5001 elements, 5001x1)]
  sprung_mass_motion.zs_PID = timeseries
  sprung_mass_motion.zs_PID.Name = 'zs_PID'
  sprung_mass_motion.zs_PID.DataInfo = tsdata.datametadata
  sprung_mass_motion.zs_PID.DataInfo.Interpolation = tsdata.interpolation
  sprung_mass_motion.zs_PID.DataInfo.Interpolation.Fhandle : function handle (value not decoded)
  sprung_mass_motion.zs_PID.DataInfo.Interpolation.Name = 'linear'
  sprung_mass_motion.zs_PID.TimeInfo = tsdata.timemetadata
  sprung_mass_motion.zs_PID.TimeInfo.Length = 5001
  sprung_mass_motion.zs_PID.TimeInfo.DuplicateTimes = 0
  sprung_mass_motion.zs_PID.TimeInfo.Increment_ = 0.001
  sprung_mass_motion.zs_PID.TimeInfo.Start_ = 0
  sprung_mass_motion.zs_PID.TimeInfo.Initialized = 1
  sprung_mass_motion.zs_PID.QualityInfo = tsdata.qualmetadata
  sprung_mass_motion.zs_PID.Data_ = [0 0 0 0 0 0 0 0 0 0 0 0 ... (5001 elements, 5001x1)]
  sprung_mass_motion.zs_passive = timeseries
  sprung_mass_motion.zs_passive.Name = 'zs_passive'
  sprung_mass_motion.zs_passive.DataInfo = tsdata.datametadata
  sprung_mass_motion.zs_passive.DataInfo.Interpolation = tsdata.interpolation
  sprung_mass_motion.zs_passive.DataInfo.Interpolation.Fhandle : function handle (value not decoded)
  sprung_mass_motion.zs_passive.DataInfo.Interpolation.Name = 'linear'
  sprung_mass_motion.zs_passive.TimeInfo = tsdata.timemetadata
  sprung_mass_motion.zs_passive.TimeInfo.Length = 5001
  sprung_mass_motion.zs_passive.TimeInfo.DuplicateTimes = 0
  sprung_mass_motion.zs_passive.TimeInfo.Increment_ = 0.001
  sprung_mass_motion.zs_passive.TimeInfo.Start_ = 0
  sprung_mass_motion.zs_passive.TimeInfo.Initialized = 1
  sprung_mass_motion.zs_passive.QualityInfo = tsdata.qualmetadata
  sprung_mass_motion.zs_passive.Data_ = [0 0 0 0 0 0 0 0 0 0 0 0 ... (5001 elements, 5001x1)]
  state_LQR.zs_zus = timeseries
  state_LQR.zs_zus.Name = 'zs_zus'
  state_LQR.zs_zus.DataInfo = tsdata.datametadata
  state_LQR.zs_zus.DataInfo.Interpolation = tsdata.interpolation
  state_LQR.zs_zus.DataInfo.Interpolation.Fhandle : function handle (value not decoded)
  state_LQR.zs_zus.DataInfo.Interpolation.Name = 'linear'
  state_LQR.zs_zus.TimeInfo = tsdata.timemetadata
  state_LQR.zs_zus.TimeInfo.Length = 5001
  state_LQR.zs_zus.TimeInfo.DuplicateTimes = 0
  state_LQR.zs_zus.TimeInfo.Increment_ = 0.001
  state_LQR.zs_zus.TimeInfo.Start_ = 0
  state_LQR.zs_zus.TimeInfo.Initialized = 1
  state_LQR.zs_zus.QualityInfo = tsdata.qualmetadata
  state_LQR.zs_zus.Data_ = [0 0 0 0 0 0 0 0 0 0 0 0 ... (5001 elements, 5001x1)]
  state_LQR.zs_d = timeseries
  state_LQR.zs_d.Name = 'zs_d'
  state_LQR.zs_d.DataInfo = tsdata.datametadata
  state_LQR.zs_d.DataInfo.Interpolation = tsdata.interpolation
  state_LQR.zs_d.DataInfo.Interpolation.Fhandle : function handle (value not decoded)
  state_LQR.zs_d.DataInfo.Interpolation.Name = 'linear'
  state_LQR.zs_d.TimeInfo = tsdata.timemetadata
  state_LQR.zs_d.TimeInfo.Length = 5001
  state_LQR.zs_d.TimeInfo.DuplicateTimes = 0
  state_LQR.zs_d.TimeInfo.Increment_ = 0.001
  state_LQR.zs_d.TimeInfo.Start_ = 0
  state_LQR.zs_d.TimeInfo.Initialized = 1
  state_LQR.zs_d.QualityInfo = tsdata.qualmetadata
  state_LQR.zs_d.Data_ = [0 0 0 0 0 0 0 0 0 0 0 0 ... (5001 elements, 5001x1)]
  state_LQR.zus_zr = timeseries
  state_LQR.zus_zr.Name = 'zus_zr'
  state_LQR.zus_zr.DataInfo = tsdata.datametadata
  state_LQR.zus_zr.DataInfo.Interpolation = tsdata.interpolation
  state_LQR.zus_zr.DataInfo.Interpolation.Fhandle : function handle (value not decoded)
  state_LQR.zus_zr.DataInfo.Interpolation.Name = 'linear'
  state_LQR.zus_zr.TimeInfo = tsdata.timemetadata
  state_LQR.zus_zr.TimeInfo.Length = 5001
  state_LQR.zus_zr.TimeInfo.DuplicateTimes = 0
  state_LQR.zus_zr.TimeInfo.Increment_ = 0.001
  state_LQR.zus_zr.TimeInfo.Start_ = 0
  state_LQR.zus_zr.TimeInfo.Initialized = 1
  state_LQR.zus_zr.QualityInfo = tsdata.qualmetadata
  state_LQR.zus_zr.Data_ = [0 0 0 0 0 0 0 0 0 0 0 0 ... (5001 elements, 5001x1)]
  state_LQR.zus_d = timeseries
  state_LQR.zus_d.Name = 'zus_d'
  state_LQR.zus_d.DataInfo = tsdata.datametadata
  state_LQR.zus_d.DataInfo.Interpolation = tsdata.interpolation
  state_LQR.zus_d.DataInfo.Interpolation.Fhandle : function handle (value not decoded)
  state_LQR.zus_d.DataInfo.Interpolation.Name = 'linear'
  state_LQR.zus_d.TimeInfo = tsdata.timemetadata
  state_LQR.zus_d.TimeInfo.Length = 5001
  state_LQR.zus_d.TimeInfo.DuplicateTimes = 0
  state_LQR.zus_d.TimeInfo.Increment_ = 0.001
  state_LQR.zus_d.TimeInfo.Start_ = 0
  state_LQR.zus_d.TimeInfo.Initialized = 1
  state_LQR.zus_d.QualityInfo = tsdata.qualmetadata
  state_LQR.zus_d.Data_ = [0 0 0 0 0 0 0 0 0 0 0 0 ... (5001 elements, 5001x1)]
  state_PID.zs_zus = timeseries
  state_PID.zs_zus.Name = 'zs_zus'
  state_PID.zs_zus.DataInfo = tsdata.datametadata
  state_PID.zs_zus.DataInfo.Interpolation = tsdata.interpolation
  state_PID.zs_zus.DataInfo.Interpolation.Fhandle : function handle (value not decoded)
  state_PID.zs_zus.DataInfo.Interpolation.Name = 'linear'
  state_PID.zs_zus.TimeInfo = tsdata.timemetadata
  state_PID.zs_zus.TimeInfo.Length = 5001
  state_PID.zs_zus.TimeInfo.DuplicateTimes = 0
  state_PID.zs_zus.TimeInfo.Increment_ = 0.001
  state_PID.zs_zus.TimeInfo.Start_ = 0
  state_PID.zs_zus.TimeInfo.Initialized = 1
  state_PID.zs_zus.QualityInfo = tsdata.qualmetadata
  state_PID.zs_zus.Data_ = [0 0 0 0 0 0 0 0 0 0 0 0 ... (5001 elements, 5001x1)]
  state_PID.zs_d = timeseries
  state_PID.zs_d.Name = 'zs_d'
  state_PID.zs_d.DataInfo = tsdata.datametadata
  state_PID.zs_d.DataInfo.Interpolation = tsdata.interpolation
  state_PID.zs_d.DataInfo.Interpolation.Fhandle : function handle (value not decoded)
  state_PID.zs_d.DataInfo.Interpolation.Name = 'linear'
  state_PID.zs_d.TimeInfo = tsdata.timemetadata
  state_PID.zs_d.TimeInfo.Length = 5001
  state_PID.zs_d.TimeInfo.DuplicateTimes = 0
  state_PID.zs_d.TimeInfo.Increment_ = 0.001
  state_PID.zs_d.TimeInfo.Start_ = 0
  state_PID.zs_d.TimeInfo.Initialized = 1
  state_PID.zs_d.QualityInfo = tsdata.qualmetadata
  state_PID.zs_d.Data_ = [0 0 0 0 0 0 0 0 0 0 0 0 ... (5001 elements, 5001x1)]
  state_PID.zus_zr = timeseries
  state_PID.zus_zr.Name = 'zus_zr'
  state_PID.zus_zr.DataInfo = tsdata.datametadata
  state_PID.zus_zr.DataInfo.Interpolation = tsdata.interpolation
  state_PID.zus_zr.DataInfo.Interpolation.Fhandle : function handle (value not decoded)
  state_PID.zus_zr.DataInfo.Interpolation.Name = 'linear'
  state_PID.zus_zr.TimeInfo = tsdata.timemetadata
  state_PID.zus_zr.TimeInfo.Length = 5001
  state_PID.zus_zr.TimeInfo.DuplicateTimes = 0
  state_PID.zus_zr.TimeInfo.Increment_ = 0.001
  state_PID.zus_zr.TimeInfo.Start_ = 0
  state_PID.zus_zr.TimeInfo.Initialized = 1
  state_PID.zus_zr.QualityInfo = tsdata.qualmetadata
  state_PID.zus_zr.Data_ = [0 0 0 0 0 0 0 0 0 0 0 0 ... (5001 elements, 5001x1)]
  state_PID.zus_d = timeseries
  state_PID.zus_d.Name = 'zus_d'
  state_PID.zus_d.DataInfo = tsdata.datametadata
  state_PID.zus_d.DataInfo.Interpolation = tsdata.interpolation
  state_PID.zus_d.DataInfo.Interpolation.Fhandle : function handle (value not decoded)
  state_PID.zus_d.DataInfo.Interpolation.Name = 'linear'
  state_PID.zus_d.TimeInfo = tsdata.timemetadata
  state_PID.zus_d.TimeInfo.Length = 5001
  state_PID.zus_d.TimeInfo.DuplicateTimes = 0
  state_PID.zus_d.TimeInfo.Increment_ = 0.001
  state_PID.zus_d.TimeInfo.Start_ = 0
  state_PID.zus_d.TimeInfo.Initialized = 1
  state_PID.zus_d.QualityInfo = tsdata.qualmetadata
  state_PID.zus_d.Data_ = [0 0 0 0 0 0 0 0 0 0 0 0 ... (5001 elements, 5001x1)]
  state_passive : object (value not decoded)
  wc_th = 3.76991118431
  wc_y = 3.76991118431
  wo_th = 18.8495559215
  wo_y = 18.8495559215
undefined symbols (not defined in the file): X, Y, Z
libraries: sm_lib x19, nesl_utility x4, slpidlib x2, slctrlblks x1, simulink x1
settings Model: Creator=omert  LastModifiedBy=omert

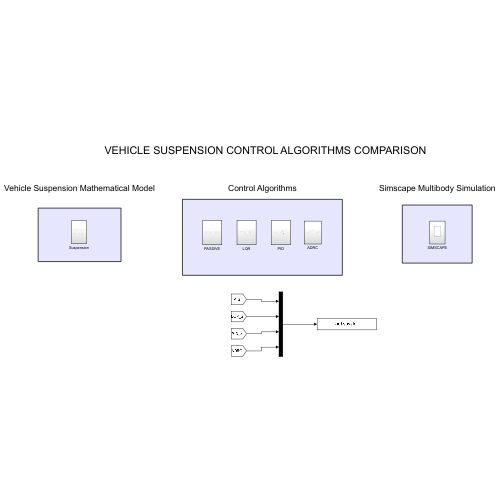
[thumbnail: Simulink's stored preview of the top-level diagram]
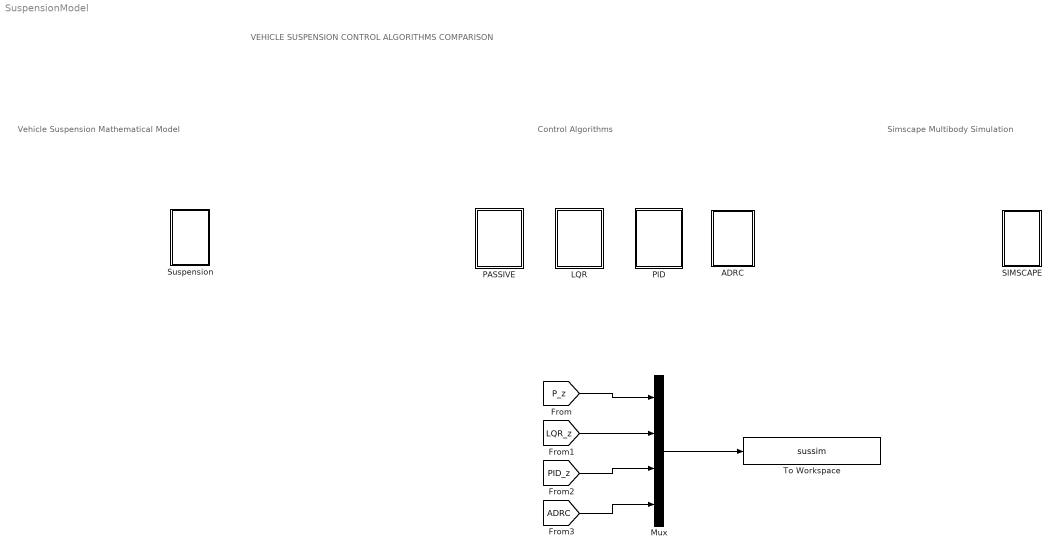
== system SuspensionModel ==
  note: VEHICLE SUSPENSION CONTROL ALGORITHMS COMPARISON
  note: Vehicle Suspension Mathematical Model
  note: Control Algorithms
  note: Simscape Multibody Simulation
  ADRC : Subsystem
  LQR : Subsystem
  Mux : Mux
  PASSIVE : Subsystem
  PID : Subsystem
  SIMSCAPE : Subsystem
  Suspension : Subsystem
  To Workspace : ToWorkspace  VariableName=sussim  SaveFormat=Structure  SampleTime=-1
  wires:
  [P_z] -> Mux/1
  [LQR_z] -> Mux/2
  [PID_z] -> Mux/3
  [ADRC] -> Mux/4
  Mux/1 -> To Workspace/1

== system SuspensionModel/ADRC ==
  Active Disturbance Rejection : slctrlblks/Active Disturbance Rejection Control  time_domain=discrete-time  Ts=0.01  model_type=second-order  b0=100  wc=1  wo=10  x0=0  ulim_checkbox=off  umax=inf  umin=-inf  xhat_checkbox=off
  Constant : Constant  Value=0
  Road Input : Subsystem
  tag scope: ADRC=global
  wires:
  Road Input/1(Out1) -> Active Disturbance Rejection/2
  Constant/1 -> Active Disturbance Rejection/1
  Active Disturbance Rejection/1 -> [ADRC]

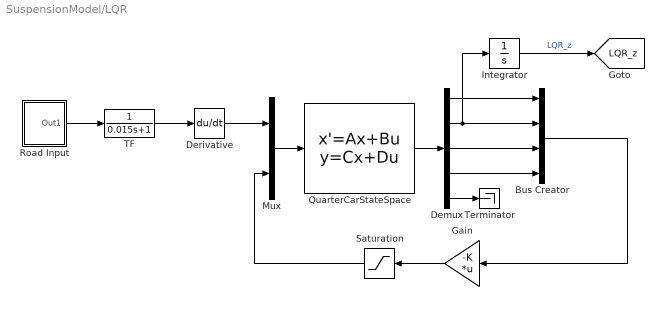
== system SuspensionModel/LQR ==
  Bus Creator : BusCreator  Inputs=4
  Demux : Demux  Outputs=5
  Derivative : Derivative
  Gain : Gain  Gain=-K  Multiplication=Matrix(K*u)
  Integrator : Integrator
  Mux : Mux  Inputs=2
  QuarterCarStateSpace : StateSpace  A=A  B=B  C=C  D=D  InitialCondition=0
  Road Input : Subsystem
  Saturation : Saturate  UpperLimit=46730  LowerLimit=-46730
  TF : TransferFcn  Denominator=[0.015 1]
  Terminator : Terminator
  tag scope: LQR_z=global
  wires:
  TF/1 -> Derivative/1
  Derivative/1 -> Mux/1
  Demux/2 -> Integrator/1, Bus Creator/2
  Bus Creator/1 -> Gain/1
  Gain/1 -> Saturation/1
  Demux/5 -> Terminator/1
  Demux/4 -> Bus Creator/4
  Demux/3 -> Bus Creator/3
  QuarterCarStateSpace/1 -> Demux/1
  Demux/1 -> Bus Creator/1
  Saturation/1 -> Mux/2
  Integrator/1 -> [LQR_z]  "LQR_z"
  Road Input/1(Out1) -> TF/1
  Mux/1 -> QuarterCarStateSpace/1

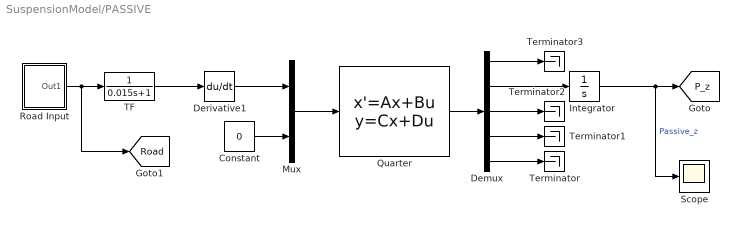
== system SuspensionModel/PASSIVE ==
  Constant : Constant  Value=0
  Demux : Demux  Outputs=5
  Derivative1 : Derivative
  Integrator : Integrator
  Mux : Mux  Inputs=2
  Quarter : StateSpace  A=A  B=B  C=C  D=D  InitialCondition=0
  Road Input : Subsystem
  Scope : Scope
  TF : TransferFcn  Denominator=[0.015 1]
  Terminator{,1..3} (4 alike) : Terminator
  tag scope: P_z=global, Road=global
  wires:
  Demux/2 -> Integrator/1
  Demux/3 -> Terminator2/1
  Integrator/1 -> Scope/1, [P_z]  "Passive_z"
  TF/1 -> Derivative1/1
  Demux/4 -> Terminator1/1
  Constant/1 -> Mux/2
  Demux/1 -> Terminator3/1
  Demux/5 -> Terminator/1
  Quarter/1 -> Demux/1
  Mux/1 -> Quarter/1
  Derivative1/1 -> Mux/1
  Road Input/1(Out1) -> [Road], TF/1

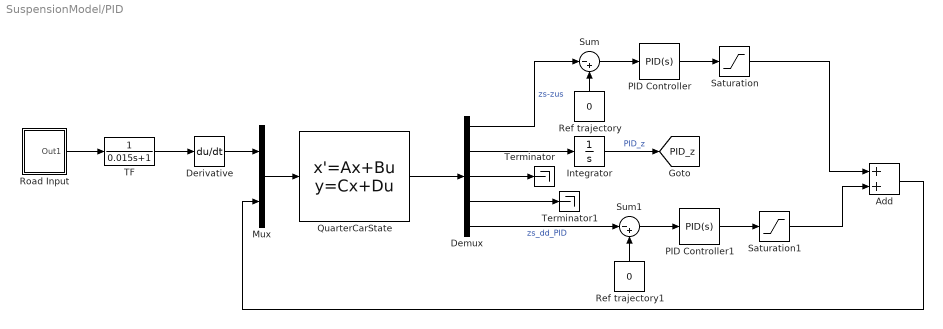
== system SuspensionModel/PID ==
  Add : Sum
  Demux : Demux  Outputs=5
  Derivative : Derivative
  Integrator : Integrator
  Mux : Mux  Inputs=2
  PID Controller : slpidlib/PID Controller  Controller=PID  Form=Parallel  TimeDomain=Continuous-time  UseExternalTs=off  SampleTime=-1  IntegratorMethod=Forward Euler  FilterMethod=Forward Euler  ControllerParametersSource=internal  P=Kp  I=Ki  UseKiTs=off  D=Kd  N=1000  UseFilter=on  TunerSelectOption=Transfer Function Based (PID Tuner App)  InitialConditionSource=internal  InitialConditionForIntegrator=0  InitialConditionForFilter=0  DifferentiatorICPrevScaledInput=0  ExternalReset=none  TrackingMode=off  Kt=1  LimitOutput=off  SatLimitsSource=internal  UpperSaturationLimit=inf  LowerSaturationLimit=-inf  LinearizeAsGain=on  AntiWindupMode=none  Kb=1  LimitIntegrator=off  UpperIntegratorSaturationLimit=inf  LowerIntegratorSaturationLimit=-inf  POutMin=[]  POutMax=[]  IOutMin=[]  IOutMax=[]  DOutMin=[]  DOutMax=[]  NOutMin=[]  NOutMax=[]  SumOutMin=[]  SumOutMax=[]  SaturationOutMin=[]  SaturationOutMax=[]  PParamMin=[]  PParamMax=[]  IParamMin=[]  IParamMax=[]  DParamMin=[]  DParamMax=[]  NParamMin=[]  NParamMax=[]  KbParamMin=[]  KbParamMax=[]  KtParamMin=[]  KtParamMax=[]  KbOutMin=[]  KbOutMax=[]  KtOutMin=[]  KtOutMax=[]  IntegratorOutMin=[]  IntegratorOutMax=[]  FilterOutMin=[]  FilterOutMax=[]  SumI1OutMin=[]  SumI1OutMax=[]  SumI2OutMin=[]  SumI2OutMax=[]  SumI3OutMin=[]  SumI3OutMax=[]  SumI4OutMin=[]  SumI4OutMax=[]  SumDOutMin=[]  SumDOutMax=[]  DifferentiatorOutMin=[]  DifferentiatorOutMax=[]  FilterDiffOutCoefMin=[]  FilterDiffOutCoefMax=[]  ReciprocalOutMin=[]  ReciprocalOutMax=[]  SumDenOutMin=[]  SumDenOutMax=[]  SumNumOutMin=[]  SumNumOutMax=[]  DivideOutMin=[]  DivideOutMax=[]  UdiffTsProdOutMin=[]  UdiffTsProdOutMax=[]  NTsProdOutMin=[]  NTsProdOutMax=[]  UintegralTsProdOutMin=[]  UintegralTsProdOutMax=[]  UngainTsProdOutMin=[]  UngainTsProdOutMax=[]  ClampingZeroOutDataTypeStr=Inherit: Inherit via back propagation  ClampingZeroOutMin=[]  ClampingZeroOutMax=[]  FilterDenConstantOutDataTypeStr=Inherit: Inherit via back propagation  FilterDenConstantOutMin=[]  FilterDenConstantOutMax=[]  PCopyOutDataTypeStr=Inherit: Inherit via back propagation  PCopyOutMin=[]  PCopyOutMax=[]  NCopyOutDataTypeStr=Inherit: Inherit via back propagation  NCopyOutMin=[]  NCopyOutMax=[]  IntegratorContinuousStateAttributes=''  IntegratorStateMustResolveToSignalObject=off  IntegratorRTWStateStorageClass=Auto  FilterContinuousStateAttributes=''  FilterStateMustResolveToSignalObject=off  FilterRTWStateStorageClass=Auto  ParallelPVariant=InternalParameters  IdealPVariant=Disabled  IVariant=InternalParameters  DVariant=InternalParameters  IntegratorVariant=Continuous  SatVariant=Disabled  AWVariant=Passthrough  PCopyVariant=Disabled  TRVariant=Disabled  FdbkBlocksVariant=Forward  IdealPFdbkVariant=Disabled  SatFdbkVariant=Disabled  DerivativeFilterVariant=ContFilter  NVariant=InternalParameters  NCopyVariant=Disabled  FilterICVariant=InternalICsFilter  IntegratorICVariant=InternalICs  ExternalResetVariant=Disabled  TRSumVariant=Passthrough  SumFdbkVariant=Disabled  SumVariant=Sum_PID  TsampFilterVariant=InternalTs  TsampNgainVariant=Passthrough  TsampIntegralVariant=Disabled_SignalSpec  ExternalSaturationOutDataTypeStr=Inherit: Same as second input
  PID Controller1 : slpidlib/PID Controller  Controller=PID  Form=Parallel  TimeDomain=Continuous-time  UseExternalTs=off  SampleTime=-1  IntegratorMethod=Forward Euler  FilterMethod=Forward Euler  ControllerParametersSource=internal  P=Kp_2  I=Ki_2  UseKiTs=off  D=Kd_2  N=1000  UseFilter=on  TunerSelectOption=Transfer Function Based (PID Tuner App)  InitialConditionSource=internal  InitialConditionForIntegrator=0  InitialConditionForFilter=0  DifferentiatorICPrevScaledInput=0  ExternalReset=none  TrackingMode=off  Kt=1  LimitOutput=off  SatLimitsSource=internal  UpperSaturationLimit=inf  LowerSaturationLimit=-inf  LinearizeAsGain=on  AntiWindupMode=none  Kb=1  LimitIntegrator=off  UpperIntegratorSaturationLimit=inf  LowerIntegratorSaturationLimit=-inf  POutMin=[]  POutMax=[]  IOutMin=[]  IOutMax=[]  DOutMin=[]  DOutMax=[]  NOutMin=[]  NOutMax=[]  SumOutMin=[]  SumOutMax=[]  SaturationOutMin=[]  SaturationOutMax=[]  PParamMin=[]  PParamMax=[]  IParamMin=[]  IParamMax=[]  DParamMin=[]  DParamMax=[]  NParamMin=[]  NParamMax=[]  KbParamMin=[]  KbParamMax=[]  KtParamMin=[]  KtParamMax=[]  KbOutMin=[]  KbOutMax=[]  KtOutMin=[]  KtOutMax=[]  IntegratorOutMin=[]  IntegratorOutMax=[]  FilterOutMin=[]  FilterOutMax=[]  SumI1OutMin=[]  SumI1OutMax=[]  SumI2OutMin=[]  SumI2OutMax=[]  SumI3OutMin=[]  SumI3OutMax=[]  SumI4OutMin=[]  SumI4OutMax=[]  SumDOutMin=[]  SumDOutMax=[]  DifferentiatorOutMin=[]  DifferentiatorOutMax=[]  FilterDiffOutCoefMin=[]  FilterDiffOutCoefMax=[]  ReciprocalOutMin=[]  ReciprocalOutMax=[]  SumDenOutMin=[]  SumDenOutMax=[]  SumNumOutMin=[]  SumNumOutMax=[]  DivideOutMin=[]  DivideOutMax=[]  UdiffTsProdOutMin=[]  UdiffTsProdOutMax=[]  NTsProdOutMin=[]  NTsProdOutMax=[]  UintegralTsProdOutMin=[]  UintegralTsProdOutMax=[]  UngainTsProdOutMin=[]  UngainTsProdOutMax=[]  ClampingZeroOutDataTypeStr=Inherit: Inherit via back propagation  ClampingZeroOutMin=[]  ClampingZeroOutMax=[]  FilterDenConstantOutDataTypeStr=Inherit: Inherit via back propagation  FilterDenConstantOutMin=[]  FilterDenConstantOutMax=[]  PCopyOutDataTypeStr=Inherit: Inherit via back propagation  PCopyOutMin=[]  PCopyOutMax=[]  NCopyOutDataTypeStr=Inherit: Inherit via back propagation  NCopyOutMin=[]  NCopyOutMax=[]  IntegratorContinuousStateAttributes=''  IntegratorStateMustResolveToSignalObject=off  IntegratorRTWStateStorageClass=Auto  FilterContinuousStateAttributes=''  FilterStateMustResolveToSignalObject=off  FilterRTWStateStorageClass=Auto  ParallelPVariant=InternalParameters  IdealPVariant=Disabled  IVariant=InternalParameters  DVariant=InternalParameters  IntegratorVariant=Continuous  SatVariant=Disabled  AWVariant=Passthrough  PCopyVariant=Disabled  TRVariant=Disabled  FdbkBlocksVariant=Forward  IdealPFdbkVariant=Disabled  SatFdbkVariant=Disabled  DerivativeFilterVariant=ContFilter  NVariant=InternalParameters  NCopyVariant=Disabled  FilterICVariant=InternalICsFilter  IntegratorICVariant=InternalICs  ExternalResetVariant=Disabled  TRSumVariant=Passthrough  SumFdbkVariant=Disabled  SumVariant=Sum_PID  TsampFilterVariant=InternalTs  TsampNgainVariant=Passthrough  TsampIntegralVariant=Disabled_SignalSpec  ExternalSaturationOutDataTypeStr=Inherit: Same as second input
  QuarterCarState : StateSpace  A=A  B=B  C=C  D=D  InitialCondition=0
  Ref trajectory : Constant  Value=0
  Ref trajectory1 : Constant  Value=0
  Road Input : Subsystem
  Saturation : Saturate  UpperLimit=46730  LowerLimit=-46730
  Saturation1 : Saturate  UpperLimit=46730  LowerLimit=-46730
  Sum : Sum  Inputs=|-+
  Sum1 : Sum  Inputs=|-+
  TF : TransferFcn  Denominator=[0.015 1]
  Terminator : Terminator
  Terminator1 : Terminator
  tag scope: PID_z=global
  wires:
  Demux/3 -> Terminator/1
  Demux/4 -> Terminator1/1
  PID Controller/1 -> Saturation/1
  Ref trajectory/1 -> Sum/2
  PID Controller1/1 -> Saturation1/1
  Demux/1 -> Sum/1  "zs-zus"
  Sum1/1 -> PID Controller1/1
  Ref trajectory1/1 -> Sum1/2
  Mux/1 -> QuarterCarState/1
  Sum/1 -> PID Controller/1
  Road Input/1(Out1) -> TF/1
  Demux/2 -> Integrator/1
  Integrator/1 -> [PID_z]  "PID_z"
  QuarterCarState/1 -> Demux/1
  TF/1 -> Derivative/1
  Derivative/1 -> Mux/1
  Add/1 -> Mux/2
  Demux/5 -> Sum1/1  "zs_dd_PID"
  Saturation1/1 -> Add/2
  Saturation/1 -> Add/1

== system SuspensionModel/SIMSCAPE ==
  PID SIMSCAPE : Subsystem

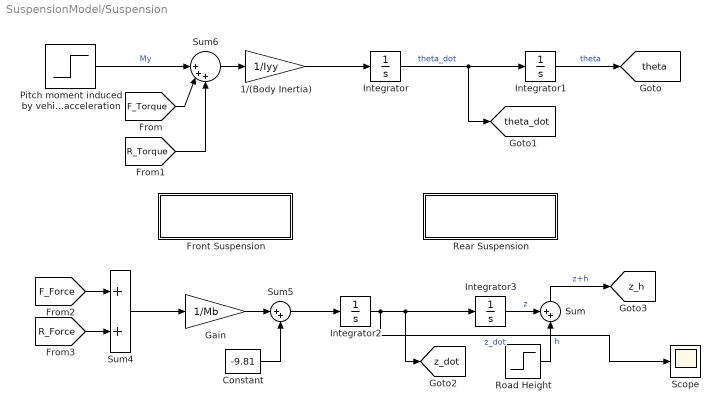
== system SuspensionModel/Suspension ==
  1/(Body Inertia) : Gain  Gain=1/Iyy  SaturateOnIntegerOverflow=on  OutDataTypeStr=Inherit: Same as input  ParamDataTypeStr=Inherit: Same as input
  Constant : Constant  Value=-9.81
  Front Suspension : Subsystem
  Gain : Gain  Gain=1/Mb  SaturateOnIntegerOverflow=on  OutDataTypeStr=Inherit: Same as input  ParamDataTypeStr=Inherit: Same as input
  Integrator : Integrator
  Integrator1 : Integrator
  Integrator2 : Integrator
  Integrator3 : Integrator  InitialCondition=-0.12
  Pitch moment induced by vehicle acceleration : Step  Time=3  After=100  SampleTime=0
  Rear Suspension : Subsystem
  Road Height : Step  Time=7  After=0.01  SampleTime=0
  Scope : Scope
  Sum : Sum  Inputs=++|
  Sum4 : Sum  InputSameDT=on  SaturateOnIntegerOverflow=on  OutDataTypeStr=Inherit: Same as first input
  Sum5 : Sum  Inputs=|++  InputSameDT=on  SaturateOnIntegerOverflow=on  OutDataTypeStr=Inherit: Same as first input
  Sum6 : Sum  Inputs=||+++  InputSameDT=on  SaturateOnIntegerOverflow=on  OutDataTypeStr=Inherit: Same as first input
  tag scope: theta=global, theta_dot=global, z_dot=global, z_h=global
  wires:
  [R_Force] -> Sum4/2
  Integrator2/1 -> Scope/1, [z_dot], Integrator3/1  "z_dot"
  Sum/1 -> [z_h]  "z+h"
  Sum5/1 -> Integrator2/1
  Integrator/1 -> [theta_dot], Integrator1/1  "theta_dot"
  Gain/1 -> Sum5/1
  [R_Torque] -> Sum6/3
  Integrator1/1 -> [theta]  "theta"
  [F_Force] -> Sum4/1
  Constant/1 -> Sum5/2
  Sum6/1 -> 1/(Body Inertia)/1
  1/(Body Inertia)/1 -> Integrator/1
  Pitch moment induced by vehicle acceleration/1 -> Sum6/1  "My"
  Sum4/1 -> Gain/1
  Integrator3/1 -> Sum/1  "z"
  [F_Torque] -> Sum6/2
  Road Height/1 -> Sum/2  "h"

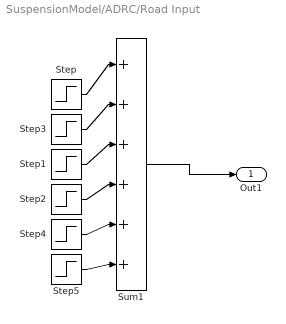
== system SuspensionModel/ADRC/Road Input ==
  Step : Step  Time=5  After=0.08  SampleTime=0
  Step1 : Step  Time=10  After=0.06  SampleTime=0
  Step2 : Step  Time=10.1  After=-0.06  SampleTime=0
  Step3 : Step  Time=5.1  After=-0.08  SampleTime=0
  Step4 : Step  Time=15  After=0.12  SampleTime=0
  Step5 : Step  Time=15.1  After=-0.12  SampleTime=0
  Sum1 : Sum  Inputs=|++++++
  Out1 : Outport
  wires:
  Step/1 -> Sum1/1
  Sum1/1 -> Out1/1
  Step3/1 -> Sum1/2
  Step5/1 -> Sum1/6
  Step4/1 -> Sum1/5
  Step2/1 -> Sum1/4
  Step1/1 -> Sum1/3

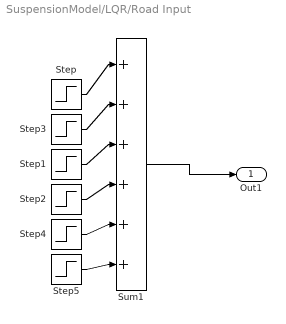
== system SuspensionModel/LQR/Road Input ==
  Step : Step  Time=5  After=0.08  SampleTime=0
  Step1 : Step  Time=10  After=0.06  SampleTime=0
  Step2 : Step  Time=10.1  After=-0.06  SampleTime=0
  Step3 : Step  Time=5.1  After=-0.08  SampleTime=0
  Step4 : Step  Time=15  After=0.12  SampleTime=0
  Step5 : Step  Time=15.1  After=-0.12  SampleTime=0
  Sum1 : Sum  Inputs=|++++++
  Out1 : Outport
  wires:
  Step/1 -> Sum1/1
  Sum1/1 -> Out1/1
  Step3/1 -> Sum1/2
  Step5/1 -> Sum1/6
  Step4/1 -> Sum1/5
  Step2/1 -> Sum1/4
  Step1/1 -> Sum1/3

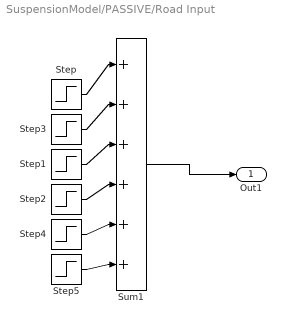
== system SuspensionModel/PASSIVE/Road Input ==
  Step : Step  Time=5  After=0.08  SampleTime=0
  Step1 : Step  Time=10  After=0.06  SampleTime=0
  Step2 : Step  Time=10.1  After=-0.06  SampleTime=0
  Step3 : Step  Time=5.1  After=-0.08  SampleTime=0
  Step4 : Step  Time=15  After=0.12  SampleTime=0
  Step5 : Step  Time=15.1  After=-0.12  SampleTime=0
  Sum1 : Sum  Inputs=|++++++
  Out1 : Outport
  wires:
  Step/1 -> Sum1/1
  Sum1/1 -> Out1/1
  Step3/1 -> Sum1/2
  Step5/1 -> Sum1/6
  Step4/1 -> Sum1/5
  Step2/1 -> Sum1/4
  Step1/1 -> Sum1/3

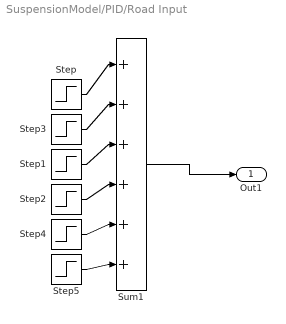
== system SuspensionModel/PID/Road Input ==
  Step : Step  Time=5  After=0.08  SampleTime=0
  Step1 : Step  Time=10  After=0.06  SampleTime=0
  Step2 : Step  Time=10.1  After=-0.06  SampleTime=0
  Step3 : Step  Time=5.1  After=-0.08  SampleTime=0
  Step4 : Step  Time=15  After=0.12  SampleTime=0
  Step5 : Step  Time=15.1  After=-0.12  SampleTime=0
  Sum1 : Sum  Inputs=|++++++
  Out1 : Outport
  wires:
  Step/1 -> Sum1/1
  Sum1/1 -> Out1/1
  Step3/1 -> Sum1/2
  Step5/1 -> Sum1/6
  Step4/1 -> Sum1/5
  Step2/1 -> Sum1/4
  Step1/1 -> Sum1/3

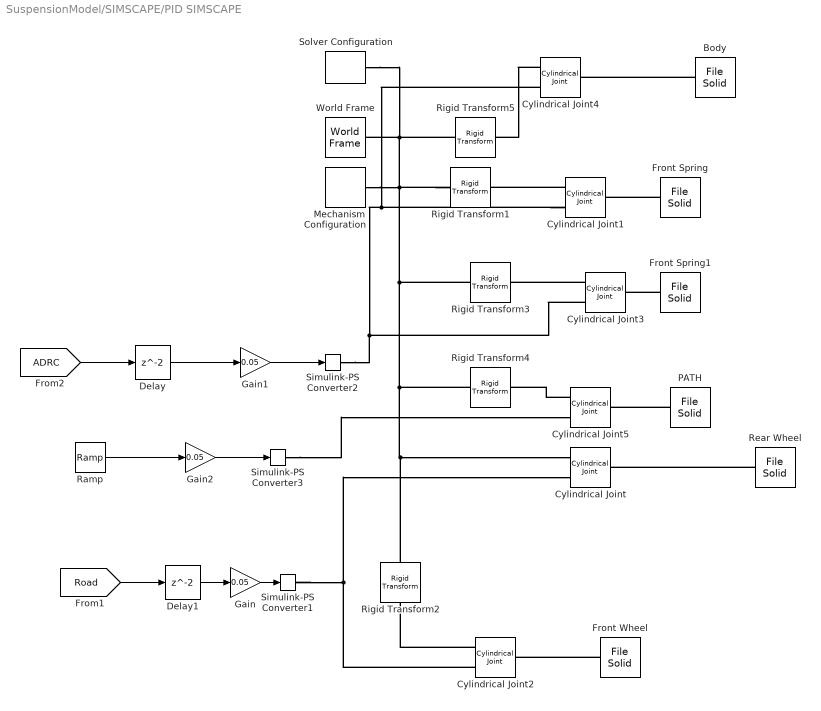
== system SuspensionModel/SIMSCAPE/PID SIMSCAPE ==
  Body : sm_lib/Body Elements/File Solid  ExtGeomFileName=C:\Users\omert\Documents\MATLAB\CyberBody.stl  UnitType=Custom  ExtGeomFileUnits=cm  StepReaderType=HEX  ExportConvexHullGeometry=off  InertiaType=Custom  Mass=1  MassUnits=kg  CenterOfMass=[0 0 0]  CenterOfMassUnits=mm  MomentsOfInertia=[1 1 1]  MomentsOfInertiaUnits=kg*mm^2  ProductsOfInertia=[0 0 0]  ProductsOfInertiaUnits=kg*mm^2  BasedOnType=Density  Density=1000  DensityUnits=kg/(m^3)  DoExposeReferenceFrame=on  SerializedFrames=<Frames/>  GraphicType=FromGeometry  MarkerShape=Sphere  MarkerSize=10  MarkerSizeUnits=m  GraphicVisPropType=SimpleVisualProperties  GraphicDiffuseColor=[0.0 0.0 0.0]  GraphicSpecularColor=[0.5 0.5 0.5 1.0]  GraphicAmbientColor=[0.15 0.15 0.15 1.0]  GraphicEmissiveColor=[0.0 0.0 0.0 1.0]  GraphicShininess=75  GraphicOpacity=0.95
  Cylindrical Joint{,1..5} (6 alike) : sm_lib/Joints/Cylindrical Joint  JointMode=Normal  SenseConstraintForce=off  SenseConstraintForceX=off  SenseConstraintForceY=off  SenseConstraintForceZ=off  SenseConstraintTorque=off  SenseConstraintTorqueX=off  SenseConstraintTorqueY=off  SenseConstraintTorqueZ=off  SenseTotalForce=off  SenseTotalForceX=off  SenseTotalForceY=off  SenseTotalForceZ=off  SenseTotalTorque=off  SenseTotalTorqueX=off  SenseTotalTorqueY=off  SenseTotalTorqueZ=off  CompositeWrenchDir=FollowerOnBase  CompositeWrenchFrame=BaseFrame  PzEquilibriumPosition=0  PzEquilibriumPositionUnits=m  PzSpringStiffness=0  PzSpringStiffnessUnits=N/m  PzDampingCoefficient=0  PzDampingCoefficientUnits=N/(m/s)  PzTorqueActuationMode=ComputedTorque  PzMotionActuationMode=InputMotion  PzSensePosition=off  PzSenseVelocity=off  PzSenseAcceleration=off  PzSenseTorqueForce=off  PzSenseLowerLimitTorqueForce=off  PzSenseUpperLimitTorqueForce=off  PzLowerLimitSpecify=off  PzLowerLimitBound=-1  PzLowerLimitBoundUnits=m  PzLowerLimitStiffness=1e6  PzLowerLimitStiffnessUnits=N/m  PzLowerLimitDamping=1e3  PzLowerLimitDampingUnits=N/(m/s)  PzLowerLimitTransitionRegionWidth=1e-4  PzLowerLimitTransitionRegionWidthUnits=m  PzUpperLimitSpecify=off  PzUpperLimitBound=1  PzUpperLimitBoundUnits=m  PzUpperLimitStiffness=1e6  PzUpperLimitStiffnessUnits=N/m  PzUpperLimitDamping=1e3  PzUpperLimitDampingUnits=N/(m/s)  PzUpperLimitTransitionRegionWidth=1e-4  PzUpperLimitTransitionRegionWidthUnits=m  PzPositionTargetSpecify=off  PzPositionTargetPriority=High  PzPositionTargetValue=0  PzPositionTargetValueUnits=m  PzVelocityTargetSpecify=off  PzVelocityTargetPriority=High  PzVelocityTargetValue=0  PzVelocityTargetValueUnits=m/s  RzEquilibriumPosition=0  RzEquilibriumPositionUnits=deg  RzSpringStiffness=0  RzSpringStiffnessUnits=N*m/deg  RzDampingCoefficient=0  RzDampingCoefficientUnits=N*m/(deg/s)  RzTorqueActuationMode=NoTorque  RzMotionActuationMode=ComputedMotion  RzSensePosition=off  RzSenseVelocity=off  RzSenseAcceleration=off  RzSenseTorqueForce=off  RzSenseLowerLimitTorqueForce=off  RzSenseUpperLimitTorqueForce=off  RzLowerLimitSpecify=off  RzLowerLimitBound=-90  RzLowerLimitBoundUnits=deg  RzLowerLimitStiffness=1e4  RzLowerLimitStiffnessUnits=N*m/deg  RzLowerLimitDamping=10  RzLowerLimitDampingUnits=N*m/(deg/s)  RzLowerLimitTransitionRegionWidth=0.1  RzLowerLimitTransitionRegionWidthUnits=deg  RzUpperLimitSpecify=off  RzUpperLimitBound=90  RzUpperLimitBoundUnits=deg  RzUpperLimitStiffness=1e4  RzUpperLimitStiffnessUnits=N*m/deg  RzUpperLimitDamping=10  RzUpperLimitDampingUnits=N*m/(deg/s)  RzUpperLimitTransitionRegionWidth=0.1  RzUpperLimitTransitionRegionWidthUnits=deg  RzPositionTargetSpecify=off  RzPositionTargetPriority=High  RzPositionTargetValue=0  RzPositionTargetValueUnits=deg  RzVelocityTargetSpecify=off  RzVelocityTargetPriority=High  RzVelocityTargetValue=0  RzVelocityTargetValueUnits=deg/s
  Delay : Delay
  Delay1 : Delay
  Front Spring : sm_lib/Body Elements/File Solid  ExtGeomFileName=C:\Users\omert\Documents\MATLAB\springv3.stl  UnitType=Custom  ExtGeomFileUnits=mm  StepReaderType=HEX  ExportConvexHullGeometry=off  InertiaType=Custom  Mass=1  MassUnits=kg  CenterOfMass=[0 0 0]  CenterOfMassUnits=mm  MomentsOfInertia=[1 1 1]  MomentsOfInertiaUnits=kg*mm^2  ProductsOfInertia=[0 0 0]  ProductsOfInertiaUnits=kg*mm^2  BasedOnType=Density  Density=1000  DensityUnits=kg/(m^3)  DoExposeReferenceFrame=on  SerializedFrames=<Frames/>  GraphicType=FromGeometry  MarkerShape=Sphere  MarkerSize=10  MarkerSizeUnits=m  GraphicVisPropType=AdvancedVisualProperties  GraphicDiffuseColor=[0.792156862745098 0.81960784313725488 0.93333333333333335]  GraphicSpecularColor=[0.5 0.5 0.5 1.0]  GraphicAmbientColor=[0.15 0.15 0.15 1.0]  GraphicEmissiveColor=[0.0 0.0 0.0 1.0]  GraphicShininess=100  GraphicOpacity=0.5
  Front Spring1 : sm_lib/Body Elements/File Solid  ExtGeomFileName=C:\Users\omert\Documents\MATLAB\springv3.stl  UnitType=Custom  ExtGeomFileUnits=mm  StepReaderType=HEX  ExportConvexHullGeometry=off  InertiaType=Custom  Mass=1  MassUnits=kg  CenterOfMass=[0 0 0]  CenterOfMassUnits=mm  MomentsOfInertia=[1 1 1]  MomentsOfInertiaUnits=kg*mm^2  ProductsOfInertia=[0 0 0]  ProductsOfInertiaUnits=kg*mm^2  BasedOnType=Density  Density=1000  DensityUnits=kg/(m^3)  DoExposeReferenceFrame=on  SerializedFrames=<Frames/>  GraphicType=FromGeometry  MarkerShape=Sphere  MarkerSize=10  MarkerSizeUnits=m  GraphicVisPropType=AdvancedVisualProperties  GraphicDiffuseColor=[0.792156862745098 0.81960784313725488 0.93333333333333335]  GraphicSpecularColor=[0.5 0.5 0.5 1.0]  GraphicAmbientColor=[0.15 0.15 0.15 1.0]  GraphicEmissiveColor=[0.0 0.0 0.0 1.0]  GraphicShininess=100  GraphicOpacity=0.5
  Front Wheel : sm_lib/Body Elements/File Solid  ExtGeomFileName=C:\Users\omert\Documents\MATLAB\CyberWheel.stl  UnitType=Custom  ExtGeomFileUnits=cm  StepReaderType=HEX  ExportConvexHullGeometry=off  InertiaType=Custom  Mass=1  MassUnits=kg  CenterOfMass=[0 0 0]  CenterOfMassUnits=mm  MomentsOfInertia=[1 1 1]  MomentsOfInertiaUnits=kg*mm^2  ProductsOfInertia=[0 0 0]  ProductsOfInertiaUnits=kg*mm^2  BasedOnType=Density  Density=1000  DensityUnits=kg/(m^3)  DoExposeReferenceFrame=on  SerializedFrames=<Frames/>  GraphicType=FromGeometry  MarkerShape=Sphere  MarkerSize=10  MarkerSizeUnits=m  GraphicVisPropType=SimpleVisualProperties  GraphicDiffuseColor=[0.0 0.0 0.0]  GraphicSpecularColor=[0.5 0.5 0.5 1.0]  GraphicAmbientColor=[0.15 0.15 0.15 1.0]  GraphicEmissiveColor=[0.0 0.0 0.0 1.0]  GraphicShininess=75  GraphicOpacity=1
  Gain : Gain  Gain=0.05
  Gain1 : Gain  Gain=0.05
  Gain2 : Gain  Gain=0.05
  Mechanism Configuration : sm_lib/Utilities/Mechanism Configuration  UniformGravity=Constant  GravityVector=[0 -0.2 0 ]  GravityVectorUnits=m/s^2  LinearizationDelta=0.001  JointModeTransitionNonlinearIterations=2
  PATH : sm_lib/Body Elements/File Solid  ExtGeomFileName=C:\Users\omert\Documents\MATLAB\p7.stl  UnitType=Custom  ExtGeomFileUnits=mm  StepReaderType=HEX  ExportConvexHullGeometry=off  InertiaType=Custom  Mass=1  MassUnits=kg  CenterOfMass=[0 0 0]  CenterOfMassUnits=mm  MomentsOfInertia=[1 1 1]  MomentsOfInertiaUnits=kg*mm^2  ProductsOfInertia=[0 0 0]  ProductsOfInertiaUnits=kg*mm^2  BasedOnType=Density  Density=1000  DensityUnits=kg/(m^3)  DoExposeReferenceFrame=on  SerializedFrames=<Frames/>  GraphicType=FromGeometry  MarkerShape=Sphere  MarkerSize=10  MarkerSizeUnits=m  GraphicVisPropType=SimpleVisualProperties  GraphicDiffuseColor=[0.0 0.0 0.0]  GraphicSpecularColor=[0.5 0.5 0.5 1.0]  GraphicAmbientColor=[0.15 0.15 0.15 1.0]  GraphicEmissiveColor=[0.0 0.0 0.0 1.0]  GraphicShininess=100  GraphicOpacity=1
  Ramp : simulink/Sources/Ramp  slope=-0.8  start=0  InitialOutput=0
  Rear Wheel : sm_lib/Body Elements/File Solid  ExtGeomFileName=C:\Users\omert\Documents\MATLAB\CyberWheel.stl  UnitType=Custom  ExtGeomFileUnits=cm  StepReaderType=HEX  ExportConvexHullGeometry=off  InertiaType=Custom  Mass=1  MassUnits=kg  CenterOfMass=[0 0 0]  CenterOfMassUnits=mm  MomentsOfInertia=[1 1 1]  MomentsOfInertiaUnits=kg*mm^2  ProductsOfInertia=[0 0 0]  ProductsOfInertiaUnits=kg*mm^2  BasedOnType=Density  Density=1000  DensityUnits=kg/(m^3)  DoExposeReferenceFrame=on  SerializedFrames=<Frames/>  GraphicType=FromGeometry  MarkerShape=Sphere  MarkerSize=10  MarkerSizeUnits=m  GraphicVisPropType=SimpleVisualProperties  GraphicDiffuseColor=[0.0 0.0 0.0]  GraphicSpecularColor=[0.5 0.5 0.5 1.0]  GraphicAmbientColor=[0.15 0.15 0.15 1.0]  GraphicEmissiveColor=[0.0 0.0 0.0 1.0]  GraphicShininess=75  GraphicOpacity=1
  Rigid Transform1 : sm_lib/Frames and Transforms/Rigid Transform  TranslationMethod=Cartesian  TranslationStandardOffset=0  TranslationStandardOffsetUnits=m  TranslationStandardAxis=+Z  TranslationCartesianOffset=[0.05167 -0.024 -0.02]  TranslationCartesianOffsetUnits=m  TranslationROffset=0  TranslationROffsetUnits=m  TranslationZOffset=0  TranslationZOffsetUnits=m  TranslationThetaOffset=0  TranslationThetaOffsetUnits=deg  RotationMethod=StandardAxis  RotationAngleUnits=deg  RotationStandardAxis=+Z  RotationAngle=0  RotationArbitraryAxis=[0 0 1]  FollAlignAxisA=+X  BaseAlignAxisA=+Y  FollAlignAxisB=+Y  BaseAlignAxisB=+Z  RotationSequenceAxes=FollowerAxes  RotationSequence=XYX  RotationSequenceAngles=[0 0 0]  RotationSequenceAnglesUnits=deg  RotationMatrix=[1 0 0; 0 1 0; 0 0 1]  Quaternion=[1 0 0 0]
  Rigid Transform2 : sm_lib/Frames and Transforms/Rigid Transform  TranslationMethod=Cartesian  TranslationStandardOffset=0  TranslationStandardOffsetUnits=m  TranslationStandardAxis=+Z  TranslationCartesianOffset=[0.097067 0 0]  TranslationCartesianOffsetUnits=m  TranslationROffset=0  TranslationROffsetUnits=m  TranslationZOffset=0  TranslationZOffsetUnits=m  TranslationThetaOffset=0  TranslationThetaOffsetUnits=deg  RotationMethod=StandardAxis  RotationAngleUnits=deg  RotationStandardAxis=+Y  RotationAngle=0  RotationArbitraryAxis=[0 0 1]  FollAlignAxisA=+X  BaseAlignAxisA=+Y  FollAlignAxisB=+Y  BaseAlignAxisB=+Z  RotationSequenceAxes=FollowerAxes  RotationSequence=XYX  RotationSequenceAngles=[0 0 0]  RotationSequenceAnglesUnits=deg  RotationMatrix=[1 0 0; 0 1 0; 0 0 1]  Quaternion=[1 0 0 0]
  Rigid Transform3 : sm_lib/Frames and Transforms/Rigid Transform  TranslationMethod=Cartesian  TranslationStandardOffset=0  TranslationStandardOffsetUnits=m  TranslationStandardAxis=+Z  TranslationCartesianOffset=[-0.04567 -0.024 -0.02]  TranslationCartesianOffsetUnits=m  TranslationROffset=0  TranslationROffsetUnits=m  TranslationZOffset=0  TranslationZOffsetUnits=m  TranslationThetaOffset=0  TranslationThetaOffsetUnits=deg  RotationMethod=StandardAxis  RotationAngleUnits=deg  RotationStandardAxis=+Z  RotationAngle=0  RotationArbitraryAxis=[0 0 1]  FollAlignAxisA=+X  BaseAlignAxisA=+Y  FollAlignAxisB=+Y  BaseAlignAxisB=+Z  RotationSequenceAxes=FollowerAxes  RotationSequence=XYX  RotationSequenceAngles=[0 0 0]  RotationSequenceAnglesUnits=deg  RotationMatrix=[1 0 0; 0 1 0; 0 0 1]  Quaternion=[1 0 0 0]
  Rigid Transform4 : sm_lib/Frames and Transforms/Rigid Transform  TranslationMethod=Cartesian  TranslationStandardOffset=0  TranslationStandardOffsetUnits=m  TranslationStandardAxis=+Z  TranslationCartesianOffset=[0.41567 -0.074 -0.032]  TranslationCartesianOffsetUnits=m  TranslationROffset=0  TranslationROffsetUnits=m  TranslationZOffset=0  TranslationZOffsetUnits=m  TranslationThetaOffset=0  TranslationThetaOffsetUnits=deg  RotationMethod=StandardAxis  RotationAngleUnits=deg  RotationStandardAxis=+Y  RotationAngle=90  RotationArbitraryAxis=[0 0 1]  FollAlignAxisA=+X  BaseAlignAxisA=+Y  FollAlignAxisB=+Y  BaseAlignAxisB=+Z  RotationSequenceAxes=FollowerAxes  RotationSequence=XYX  RotationSequenceAngles=[0 0 0]  RotationSequenceAnglesUnits=deg  RotationMatrix=[1 0 0; 0 1 0; 0 0 1]  Quaternion=[1 0 0 0]
  Rigid Transform5 : sm_lib/Frames and Transforms/Rigid Transform  TranslationMethod=None  TranslationStandardOffset=0  TranslationStandardOffsetUnits=m  TranslationStandardAxis=+Z  TranslationCartesianOffset=[0 0 0]  TranslationCartesianOffsetUnits=m  TranslationROffset=0  TranslationROffsetUnits=m  TranslationZOffset=0  TranslationZOffsetUnits=m  TranslationThetaOffset=0  TranslationThetaOffsetUnits=deg  RotationMethod=StandardAxis  RotationAngleUnits=deg  RotationStandardAxis=+Z  RotationAngle=0  RotationArbitraryAxis=[0 0 1]  FollAlignAxisA=+X  BaseAlignAxisA=+Y  FollAlignAxisB=+Y  BaseAlignAxisB=+Z  RotationSequenceAxes=FollowerAxes  RotationSequence=XYX  RotationSequenceAngles=[0 0 0]  RotationSequenceAnglesUnits=deg  RotationMatrix=[1 0 0; 0 1 0; 0 0 1]  Quaternion=[1 0 0 0]
  Simulink-PS Converter1 : nesl_utility/Simulink-PS Converter  PhysicalDomain=network_engine_domain  SubClassName=ps_input  LeftPortType=input  RightPortType=output  PseudoPeriodic=off  Frequencies=[]  NoiseDistribution=none  NoiseParameters=[]  Unit=1  AffineConversion=off  FilteringAndDerivatives=filter  SimscapeFilterOrder=2  InputFilterTimeConstant=0.001  UdotUserProvided=0
  Simulink-PS Converter2 : nesl_utility/Simulink-PS Converter  PhysicalDomain=network_engine_domain  SubClassName=ps_input  LeftPortType=input  RightPortType=output  PseudoPeriodic=off  Frequencies=[]  NoiseDistribution=none  NoiseParameters=[]  Unit=1  AffineConversion=off  FilteringAndDerivatives=filter  SimscapeFilterOrder=2  InputFilterTimeConstant=0.001  UdotUserProvided=0
  Simulink-PS Converter3 : nesl_utility/Simulink-PS Converter  PhysicalDomain=network_engine_domain  SubClassName=ps_input  LeftPortType=input  RightPortType=output  PseudoPeriodic=off  Frequencies=[]  NoiseDistribution=none  NoiseParameters=[]  Unit=1  AffineConversion=off  FilteringAndDerivatives=filter  SimscapeFilterOrder=2  InputFilterTimeConstant=0.001  UdotUserProvided=0
  Solver Configuration : nesl_utility/Solver Configuration  PhysicalDomain=network_engine_domain  SubClassName=solver  LeftPortType=input  RightPortType=generic  Tones=[]  Harmonics=[]  SimulateNoise=off  Profile=off  UseLocalSampling=off  EnableSwitchedLinearOptims=on  FrequencyDomain=off  UseCCode=off  RelTol=0.001  AbsTol=1e-06  MinStep=1e-09  ToWorkspace=off  RevertToSquareIcSolve=off  NumHomotopyIterations=100  PhasorMode=off  PhasorModeNumHarmonics=1  ConsistencySolver=NEWTON_FTOL  IndexReductionMethod=DerivativeReplacement  DoDC=off  ResidualTolerance=1e-04  ConsistencyTolSource=GLOBAL  ConsistencyAbsTol=0.001  ConsistencyRelTol=0.001  ConsistencyTolFactor=0.001  UseLocalSolver=off  LocalSolverChoice=NE_BACKWARD_EULER_ADVANCER  ResolveIndetEquations=on  FunctionEvalNumThread=1  LocalSolverSampleTime=0.001  DoFixedCost=off  MaxNonlinIter=3  MaxModeIter=2  ComputeImpulses=off  ImpulseIterations=2  LinearAlgebra=Sparse  LinearAlgebraNumThread=0  EquationFormulation=NE_TIME_EF  DelaysMemoryBudget=1024  AutomaticFiltering=on  FilteringTimeConstant=0.001  PartitionStorageMethod=AS_NEEDED  PartitionMemoryBudget=1024  PartitionMethod=FAST
  World Frame : sm_lib/Frames and Transforms/World Frame
  wires:
  Gain/1 -> Simulink-PS Converter1/1
  Gain1/1 -> Simulink-PS Converter2/1
  [Road] -> Delay1/1
  Gain2/1 -> Simulink-PS Converter3/1
  Ramp/1 -> Gain2/1
  Delay/1 -> Gain1/1
  Delay1/1 -> Gain/1
  [ADRC] -> Delay/1
  connections:
  Cylindrical Joint2/LConn1 -- Rigid Transform2/RConn1
  Cylindrical Joint1/LConn1 -- Rigid Transform1/RConn1
  Simulink-PS Converter2/RConn1 -- Cylindrical Joint4/LConn2 -- Cylindrical Joint1/LConn2 -- Cylindrical Joint3/LConn2
  Front Wheel/RConn1 -- Cylindrical Joint2/RConn1
  Cylindrical Joint3/LConn1 -- Rigid Transform3/RConn1
  Front Spring1/RConn1 -- Cylindrical Joint3/RConn1
  Cylindrical Joint4/LConn1 -- Rigid Transform5/RConn1
  Simulink-PS Converter1/RConn1 -- Cylindrical Joint/LConn2 -- Cylindrical Joint2/LConn2
  Body/RConn1 -- Cylindrical Joint4/RConn1
  Front Spring/RConn1 -- Cylindrical Joint1/RConn1
  Simulink-PS Converter3/RConn1 -- Cylindrical Joint5/LConn2
  Cylindrical Joint5/LConn1 -- Rigid Transform4/RConn1
  PATH/RConn1 -- Cylindrical Joint5/RConn1
  Rigid Transform5/LConn1 -- Solver Configuration/RConn1 -- Rigid Transform2/LConn1 -- Cylindrical Joint/LConn1 -- Rigid Transform4/LConn1 -- Rigid Transform3/LConn1 -- Rigid Transform1/LConn1 -- Mechanism Configuration/RConn1 -- World Frame/RConn1
  Rear Wheel/RConn1 -- Cylindrical Joint/RConn1

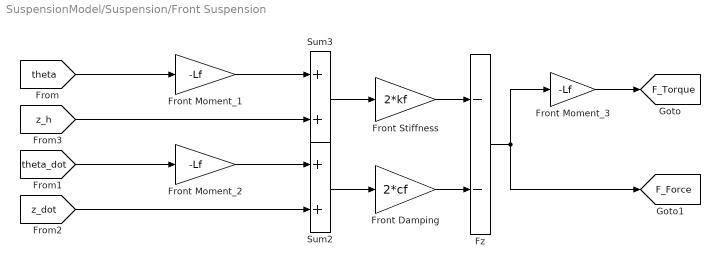
== system SuspensionModel/Suspension/Front Suspension ==
  Front Damping : Gain  Gain=2*cf  SaturateOnIntegerOverflow=on  OutDataTypeStr=Inherit: Same as input  ParamDataTypeStr=Inherit: Same as input
  Front Moment_1 : Gain  Gain=-Lf  SaturateOnIntegerOverflow=on  OutDataTypeStr=Inherit: Same as input  ParamDataTypeStr=Inherit: Same as input
  Front Moment_2 : Gain  Gain=-Lf  SaturateOnIntegerOverflow=on  OutDataTypeStr=Inherit: Same as input  ParamDataTypeStr=Inherit: Same as input
  Front Moment_3 : Gain  Gain=-Lf  SaturateOnIntegerOverflow=on  OutDataTypeStr=Inherit: Same as input  ParamDataTypeStr=Inherit: Same as input
  Front Stiffness : Gain  Gain=2*kf  SaturateOnIntegerOverflow=on  OutDataTypeStr=Inherit: Same as input  ParamDataTypeStr=Inherit: Same as input
  Fz : Sum  Inputs=--  InputSameDT=on  SaturateOnIntegerOverflow=on  OutDataTypeStr=Inherit: Same as first input
  Sum2 : Sum  InputSameDT=on  SaturateOnIntegerOverflow=on  OutDataTypeStr=Inherit: Same as first input
  Sum3 : Sum  InputSameDT=on  SaturateOnIntegerOverflow=on  OutDataTypeStr=Inherit: Same as first input
  tag scope: F_Force=global, F_Torque=global
  wires:
  [theta_dot] -> Front Moment_2/1
  Fz/1 -> [F_Force], Front Moment_3/1
  [z_dot] -> Sum2/2
  Front Moment_3/1 -> [F_Torque]
  Front Moment_2/1 -> Sum2/1
  Front Damping/1 -> Fz/2
  [theta] -> Front Moment_1/1
  [z_h] -> Sum3/2
  Front Moment_1/1 -> Sum3/1
  Sum2/1 -> Front Damping/1
  Sum3/1 -> Front Stiffness/1
  Front Stiffness/1 -> Fz/1

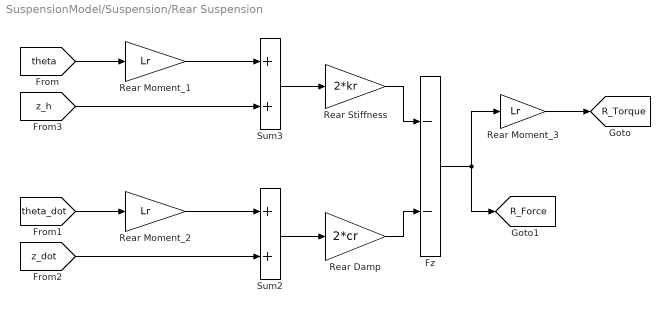
== system SuspensionModel/Suspension/Rear Suspension ==
  Fz : Sum  Inputs=--  InputSameDT=on  SaturateOnIntegerOverflow=on  OutDataTypeStr=Inherit: Same as first input
  Rear Damp : Gain  Gain=2*cr  SaturateOnIntegerOverflow=on  OutDataTypeStr=Inherit: Same as input  ParamDataTypeStr=Inherit: Same as input
  Rear Moment_1 : Gain  Gain=Lr  SaturateOnIntegerOverflow=on  OutDataTypeStr=Inherit: Same as input  ParamDataTypeStr=Inherit: Same as input
  Rear Moment_2 : Gain  Gain=Lr  SaturateOnIntegerOverflow=on  OutDataTypeStr=Inherit: Same as input  ParamDataTypeStr=Inherit: Same as input
  Rear Moment_3 : Gain  Gain=Lr  SaturateOnIntegerOverflow=on  OutDataTypeStr=Inherit: Same as input  ParamDataTypeStr=Inherit: Same as input
  Rear Stiffness : Gain  Gain=2*kr  SaturateOnIntegerOverflow=on  OutDataTypeStr=Inherit: Same as input  ParamDataTypeStr=Inherit: Same as input
  Sum2 : Sum  InputSameDT=on  SaturateOnIntegerOverflow=on  OutDataTypeStr=Inherit: Same as first input
  Sum3 : Sum  InputSameDT=on  SaturateOnIntegerOverflow=on  OutDataTypeStr=Inherit: Same as first input
  tag scope: R_Force=global, R_Torque=global
  wires:
  Fz/1 -> [R_Force], Rear Moment_3/1
  Sum2/1 -> Rear Damp/1
  Rear Moment_1/1 -> Sum3/1
  [theta] -> Rear Moment_1/1
  Rear Moment_3/1 -> [R_Torque]
  [z_dot] -> Sum2/2
  Sum3/1 -> Rear Stiffness/1
  Rear Moment_2/1 -> Sum2/1
  Rear Stiffness/1 -> Fz/1
  [z_h] -> Sum3/2
  Rear Damp/1 -> Fz/2
  [theta_dot] -> Rear Moment_2/1
